simulink model "43_BusNetworkElectricityTransmissionModel"  (R2023b)
settings: Solver=VariableStepAuto  StartTime=0.0  StopTime=0.8  RelTol=1e-3
model workspace (MAT data in the model file):
  BESS_Fp_KDroop = 0.025
  BESS_KSI = 817
  BESS_PWM_fs = 560
  BESS_P_Ki = 0.5
  BESS_P_Kp = 0.0636
  BESS_Pnom = 3000000
  BESS_Q_Ki = 1
  BESS_Q_Kp = 0.0257
  BESS_Vd_Ki = 850
  BESS_Vd_Kp = 0.216
  BESS_Vnom = 1000
  BESS_Vq_KDroop = 0.025
  BESS_Vq_Ki = 850
  BESS_Vq_Kp = 0.216
  Compensation_Ki = 30
  Compensation_Kp = 3
  DC_Ki = 400
  DC_Kp = 8
  F = 0.01
  Flux_min = 0.5
  Grid_Freq_PWM = 2700
  Grid_Ireg_Ki = 5
  Grid_Ireg_Kp = 0.83
  Grid_Ireg_lim = 1.1
  Grid_Modindex_Upper = 1.1
  Grid_conv_Imax = 0.8
  H = 0.685
  Idref_max = 0.9
  Iqref_Tc = 0.3
  Ki_Var = 0.05
  Ki_Vreg = 20
  Ksh = 1.1
  L_pu = 0.3
  Llr = 0.16
  Lls = 0.18
  Lm = 2.9
  LowLoad_P = 130
  Nb_wt = 6
  P_mech = 1080000
  PeakShav_P = 200
  Pitch_Ki = 0
  Pitch_Kp = 150
  Pitch_Max = 27
  Pitch_Tc = 0.01
  Pitch_rate = 10
  Q_Filt = 50
  R_pu = 0.003
  Rotor_Freq_PWM = 1620
  Rotor_Ireg_Ki = 8
  Rotor_Ireg_Kp = 0.6
  Rotor_Ireg_lim = 0.1
  Rotor_Modindex_Upper = 2
  Rr = 0.016
  Rs = 0.023
  SOCBESS : Simulink.Parameter (value not decoded)
  T_set = 0.0001
  Tp = 5e-05
  Ts = 5e-06
  Var_C_Filt = 720000
  Var_reg_max = 1.1
  Var_reg_min = 0.9
  WT_Coeff = [0.645 116 0.4 5 21 0.00912 0.08 0.035]
  WT_H = 4.32
  WT_IGBTRon = 5.931
  WT_Param = [91.204 10143]
  Wind_Freq_Filt = 10000
  Wind_Freq_nom = 60
  Wind_P_nom = 1200000
  Wind_Rotor_V_nom = 1950
  Wind_V_nom = 500
  Zeta_Filt = 0.707106781187
  init = [-0.2 0 0 0 0 0 0 0]
  p = 3
  torque0 = 0.83
  v_Ki = 0.1
  v_Kp = 3.6
  v_Max = 1.2
  v_Min = 0.7
  v_T = 5
  vreg_max = 1
  wind_VDC_nom = 1150
  wt0 = 1.2
undefined symbols (not defined in the file): D1, D11, Delta, DiscIntNeverNeededParam, Iabc, Ion, Lithium, P, Q, Vabc
libraries: powerlib_extras x156, spsSeriesRLCBranchLib x66, spsLoadFlowBusLib x43, spsThreePhaseSeriesRLCLoadLib x33, spsThreePhaseTransformerTwoWindingsLib x32, spsThreePhaseVIMeasurementLib x30, simulink_extras x30, spsDistributedParametersLineLib x22, spsGenericPowerSystemStabilizerLib x20, spsSynchronousMachinepuStandardLib x10, spsExcitationSystemLib x10, spsHydraulicTurbineandGovernorLib x10
(part 5 of 19)

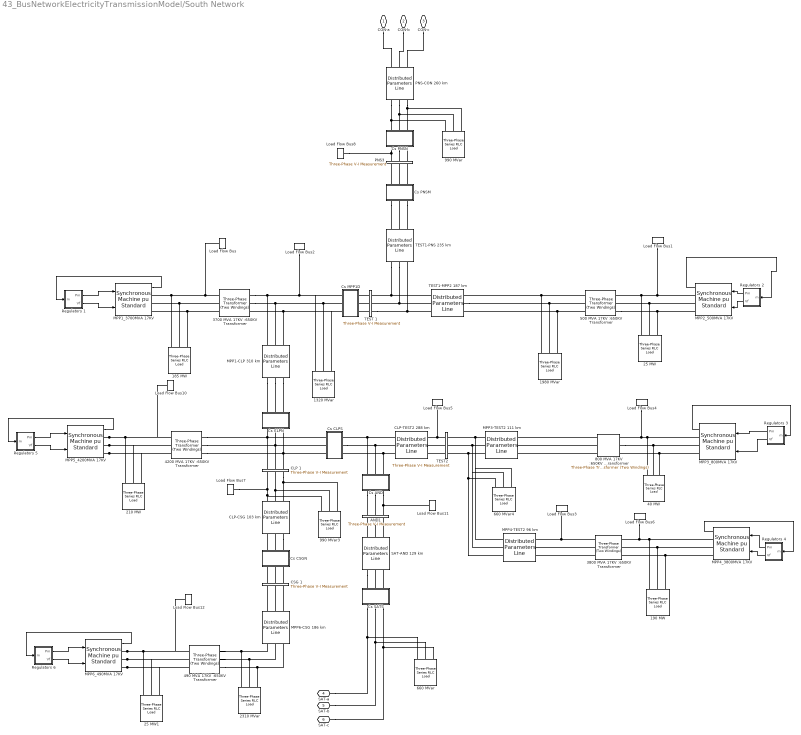
== system 43_BusNetworkElectricityTransmissionModel/South Network ==
  " SAT-AND 129 km" : spsDistributedParametersLineLib/Distributed Parameters Line  Phases=3  Length=129  Frequency=60  Resistance=[0.01273 0.3864]/6  Inductance="[0.9337e-3  4.1264e-3]/6"  Capacitance=[12.74e-9 7.751e-9]*6  x1=[-0.00078 2.60302457371263e-08 -160778.939869371 -239310.302920162;-0.00072 2.65712134423961e-08 -155325.195833165 -242885.5399717;-0.00066 2.70985868238892e-08 -149791.98455669 -246336.512292981;-0.0006 2.76120960676389e-08 -144182.136933079 -249661.454302796;-0.00054 2.81114784528276e-08 -138498.523064033 -252858.664899377;-0.00048 2.85964784861993e-08 -132744.050791429 -255926.508330705;-0.00042 2.90668480327754e-08 -126921.664209612 -258863.415031392;-0.00036 2.95223464428043e-08 -121034.342159143 -261667.882425704;-0.0003 2.99627406748828e-08 -115085.096702768 -264338.4756963;-0.00024 3.03878054151842e-08 -109076.971584392 -266873.828518316;-0.00018 3.07973231927332e-08 -103013.040671842 -269272.643758401;-0.00012 3.11910844906677e-08 -96896.4063842224 -271533.694138353;-6e-05 3.15688878534317e-08 -90730.1981046569 -273655.822863018]  x2=[-0.00078 5.55178195316479e-08 -88962.2973602101 -231944.533349288;-0.00072 5.76982364407432e-08 -83693.5243512018 -233897.335995697;-0.00066 5.98491338659346e-08 -78381.9321886569 -235730.472443085;-0.0006 6.19694113683554e-08 -73030.2383812726 -237443.004824972;-0.00054 6.4057984174857e-08 -67641.1809544889 -239034.056978149;-0.00048 6.61137837329993e-08 -62217.5170496635 -240502.814890934;-0.00042 6.81357582577416e-08 -56762.021513468 -241848.52711964;-0.00036 7.01228732695551e-08 -51277.4854782247 -243070.505173024;-0.0003 7.20741121236823e-08 -45766.7149339116 -244168.123864536;-0.00024 7.39884765302704e-08 -40232.5292925668 -245140.82163217;-0.00018 7.58649870651158e-08 -34677.7599458242 -245988.100825776;-0.00012 7.7702683670755e-08 -29105.2488163219 -246709.527961661;-6e-05 7.95006261476476e-08 -23517.8469037221 -247304.733944374]  x3=[-0.00078 -1.62971978119486e-09 -2676.70735567061 -14439.1653842091;-0.00072 -1.59483091706544e-09 -2349.44448965774 -14496.0134442237;-0.00066 -1.55912610796977e-09 -2020.97960443123 -14545.4450759047;-0.0006 -1.52262362114792e-09 -1691.48074869568 -14587.4349891159;-0.00054 -1.48534213194664e-09 -1361.11650015412 -14621.9617010419;-0.00048 -1.4473007142647e-09 -1030.05587926054 -14649.0075471789;-0.00042 -1.40851883079429e-09 -698.468262745896 -14668.5586903722;-0.00036 -1.36901632306361e-09 -366.523296961816 -14680.6051278957;-0.0003 -1.32881340128554e-09 -34.3908110864396 -14685.1406965693;-0.00024 -1.28793063401772e-09 297.759269763359 -14682.1630759124;-0.00018 -1.24638893763932e-09 629.757011468787 -14671.6737893307;-0.00012 -1.2042095656498e-09 961.432557850576 -14653.678203337;-6e-05 -1.16141409779526e-09 1292.61621757054 -14628.1855248057]  x4=[-0.00078 2.13998612808817e-09 -3708.50494908711 4506.04674626499;-0.00072 2.12843326610419e-09 -3809.4714718435 4421.01671562987;-0.00066 2.11579145833235e-09 -3908.48899860396 4333.72481115204;-0.0006 2.1020671725551e-09 -4005.50687017216 4244.2156929828;-0.00054 2.08726743037064e-09 -4100.47545041233 4152.53515564094;-0.00048 2.07139980360052e-09 -4193.34615164399 4058.73010458342;-0.00042 2.05447241041582e-09 -4284.07145950033 3962.84853220769;-0.00036 2.03649391118366e-09 -4372.60495723746 3864.93949329786;-0.0003 2.01747350403647e-09 -4458.90134948202 3765.05307992739;-0.00024 1.99742092016598e-09 -4542.91648540516 3663.24039583105;-0.00018 1.97634641884464e-09 -4624.60738131092 3559.5535302593;-0.00012 1.95426078217673e-09 -4703.93224262748 3454.04553132848;-6e-05 1.93117530958208e-09 -4780.85048529004 3346.77037888041]  x5=0.000729548621424508  V1=[2.188e-18 3.182e-07 3.182e-07;377 377 377;0.6306 1.295 -0.2758]  V2=[1.209e-19 1.011e-07 1.011e-07;377 377 377;-2.255 -1.798 2.915]  I1=[1.016e-20 9.164e-09 9.164e-09;377 377 377;2.19 2.786 1.215]  I2=[1.089e-20 9.22e-09 9.22e-09;377 377 377;-0.7019 -0.2685 -1.839]  nHarmo=1  Measurements=None  Decoupling=off  VsMag0=0  VrMag0=0  VsAngle0=0  VrAngle0=0  IsMag0=0  IrMag0=0  IsAngle0=0  IrAngle0=0
      settings: LibrarySourceBlock=sps_lib/Power Grid Elements/Distributed Parameters Line
  1320 MVar : spsThreePhaseSeriesRLCLoadLib/Three-Phase Series RLC Load  LConnTagsString=A|B|C  Configuration=Y (grounded)  NominalVoltage=650e3  Vabc=[1e3 1e3 1e3]  Vabcp=[1e3 1e3 1e3]  NominalFrequency=60  UnbalancedPower=off  ActivePower=4400e3  InductivePower=1320e6  CapacitivePower=0  Pabc=[10e3 9e3 11e3]  QLabc=[100 90 110]  QCabc=[100 90 110]  Pabcp=[10e3 9e3 11e3]  QLabcp=[100 90 110]  QCabcp=[100 90 110]  Measurements=None  LoadType=constant Z
  185 MW : spsThreePhaseSeriesRLCLoadLib/Three-Phase Series RLC Load  LConnTagsString=A|B|C  Configuration=Y (grounded)  NominalVoltage=17e3  Vabc=[1e3 1e3 1e3]  Vabcp=[1e3 1e3 1e3]  NominalFrequency=60  UnbalancedPower=off  ActivePower=185e6  InductivePower=0  CapacitivePower=0  Pabc=[10e3 9e3 11e3]  QLabc=[100 90 110]  QCabc=[100 90 110]  Pabcp=[10e3 9e3 11e3]  QLabcp=[100 90 110]  QCabcp=[100 90 110]  Measurements=None  LoadType=constant Z
  190 MW : spsThreePhaseSeriesRLCLoadLib/Three-Phase Series RLC Load  LConnTagsString=A|B|C  Configuration=Y (grounded)  NominalVoltage=17e3  Vabc=[1e3 1e3 1e3]  Vabcp=[1e3 1e3 1e3]  NominalFrequency=60  UnbalancedPower=off  ActivePower=190e6  InductivePower=0  CapacitivePower=0  Pabc=[10e3 9e3 11e3]  QLabc=[100 90 110]  QCabc=[100 90 110]  Pabcp=[10e3 9e3 11e3]  QLabcp=[100 90 110]  QCabcp=[100 90 110]  Measurements=None  LoadType=constant Z
  1980 MVar : spsThreePhaseSeriesRLCLoadLib/Three-Phase Series RLC Load  LConnTagsString=A|B|C  Configuration=Y (grounded)  NominalVoltage=650e3  Vabc=[1e3 1e3 1e3]  Vabcp=[1e3 1e3 1e3]  NominalFrequency=60  UnbalancedPower=off  ActivePower=4400e3  InductivePower=1320e6  CapacitivePower=0  Pabc=[10e3 9e3 11e3]  QLabc=[100 90 110]  QCabc=[100 90 110]  Pabcp=[10e3 9e3 11e3]  QLabcp=[100 90 110]  QCabcp=[100 90 110]  Measurements=None  LoadType=constant Z
  210 MW : spsThreePhaseSeriesRLCLoadLib/Three-Phase Series RLC Load  LConnTagsString=A|B|C  Configuration=Y (grounded)  NominalVoltage=17e3  Vabc=[1e3 1e3 1e3]  Vabcp=[1e3 1e3 1e3]  NominalFrequency=60  UnbalancedPower=off  ActivePower=210e6  InductivePower=0  CapacitivePower=0  Pabc=[10e3 9e3 11e3]  QLabc=[100 90 110]  QCabc=[100 90 110]  Pabcp=[10e3 9e3 11e3]  QLabcp=[100 90 110]  QCabcp=[100 90 110]  Measurements=None  LoadType=constant Z
  2310 MVar : spsThreePhaseSeriesRLCLoadLib/Three-Phase Series RLC Load  LConnTagsString=A|B|C  Configuration=Y (grounded)  NominalVoltage=650e3  Vabc=[1e3 1e3 1e3]  Vabcp=[1e3 1e3 1e3]  NominalFrequency=60  UnbalancedPower=off  ActivePower=7700e3  InductivePower=2310e6  CapacitivePower=0  Pabc=[10e3 9e3 11e3]  QLabc=[100 90 110]  QCabc=[100 90 110]  Pabcp=[10e3 9e3 11e3]  QLabcp=[100 90 110]  QCabcp=[100 90 110]  Measurements=None  LoadType=constant Z
  25 MW : spsThreePhaseSeriesRLCLoadLib/Three-Phase Series RLC Load  LConnTagsString=A|B|C  Configuration=Y (grounded)  NominalVoltage=17e3  Vabc=[1e3 1e3 1e3]  Vabcp=[1e3 1e3 1e3]  NominalFrequency=60  UnbalancedPower=off  ActivePower=25e6  InductivePower=0  CapacitivePower=0  Pabc=[10e3 9e3 11e3]  QLabc=[100 90 110]  QCabc=[100 90 110]  Pabcp=[10e3 9e3 11e3]  QLabcp=[100 90 110]  QCabcp=[100 90 110]  Measurements=None  LoadType=constant Z
  25 MW1 : spsThreePhaseSeriesRLCLoadLib/Three-Phase Series RLC Load  LConnTagsString=A|B|C  Configuration=Y (grounded)  NominalVoltage=17e3  Vabc=[1e3 1e3 1e3]  Vabcp=[1e3 1e3 1e3]  NominalFrequency=60  UnbalancedPower=off  ActivePower=25e6  InductivePower=0  CapacitivePower=0  Pabc=[10e3 9e3 11e3]  QLabc=[100 90 110]  QCabc=[100 90 110]  Pabcp=[10e3 9e3 11e3]  QLabcp=[100 90 110]  QCabcp=[100 90 110]  Measurements=None  LoadType=constant Z
  "3700 MVA 17KV :650KV Transformer " : spsThreePhaseTransformerTwoWindingsLib/Three-Phase Transformer (Two Windings)  Winding1Connection=Delta (D1)  Winding2Connection=Yg  CoreType=Three single-phase transformers  SetSaturation=off  Hysteresis=off  DataFile='hysteresis'  SetInitialFlux=off  Measurements=None  UNITS=pu  NominalPower=[ 3700e6 , 60 ]  Winding1=[ 17e3 , 0.002 , 0.08 ]  Winding2=[ 650e3 , 0.002 , 0.08 ]  Rm=500  Lm=500  L0=0.5  Saturation=[ 0,0 ; 0.0024,1.2 ; 1.0,1.52 ]  InitialFluxes=[ 0.8 , -0.8 , 0.7 ]  BreakLoop=off  DiscreteSolver=Trapezoidal iterative  DataType=off  TransfoNumber=1
  3800 MVA 17KV :650KV Transformer : spsThreePhaseTransformerTwoWindingsLib/Three-Phase Transformer (Two Windings)  Winding1Connection=Yg  Winding2Connection=Delta (D1)  CoreType=Three single-phase transformers  SetSaturation=off  Hysteresis=off  DataFile='hysteresis'  SetInitialFlux=off  Measurements=None  UNITS=pu  NominalPower=[ 3800e6 , 60 ]  Winding1=[ 650e3 , 0.002 , 0.08 ]  Winding2=[ 17e3 , 0.002 , 0.08 ]  Rm=500  Lm=500  L0=0.5  Saturation=[ 0,0 ; 0.0024,1.2 ; 1.0,1.52 ]  InitialFluxes=[ 0.8 , -0.8 , 0.7 ]  BreakLoop=off  DiscreteSolver=Trapezoidal iterative  DataType=off  TransfoNumber=1
  40 MW : spsThreePhaseSeriesRLCLoadLib/Three-Phase Series RLC Load  LConnTagsString=A|B|C  Configuration=Y (grounded)  NominalVoltage=17e3  Vabc=[1e3 1e3 1e3]  Vabcp=[1e3 1e3 1e3]  NominalFrequency=60  UnbalancedPower=off  ActivePower=40e6  InductivePower=0  CapacitivePower=0  Pabc=[10e3 9e3 11e3]  QLabc=[100 90 110]  QCabc=[100 90 110]  Pabcp=[10e3 9e3 11e3]  QLabcp=[100 90 110]  QCabcp=[100 90 110]  Measurements=None  LoadType=constant Z
  4200 MVA 17KV :650KV Transformer : spsThreePhaseTransformerTwoWindingsLib/Three-Phase Transformer (Two Windings)  Winding1Connection=Delta (D1)  Winding2Connection=Yg  CoreType=Three single-phase transformers  SetSaturation=off  Hysteresis=off  DataFile='hysteresis'  SetInitialFlux=off  Measurements=None  UNITS=pu  NominalPower=[ 4200e6 , 60 ]  Winding1=[ 17e3 , 0.002 , 0.08 ]  Winding2=[ 650e3 , 0.002 , 0.08 ]  Rm=500  Lm=500  L0=0.5  Saturation=[ 0,0 ; 0.0024,1.2 ; 1.0,1.52 ]  InitialFluxes=[ 0.8 , -0.8 , 0.7 ]  BreakLoop=off  DiscreteSolver=Trapezoidal iterative  DataType=off  TransfoNumber=1
  490 MVA 17KV :650KV Transformer : spsThreePhaseTransformerTwoWindingsLib/Three-Phase Transformer (Two Windings)  Winding1Connection=Delta (D1)  Winding2Connection=Yg  CoreType=Three single-phase transformers  SetSaturation=off  Hysteresis=off  DataFile='hysteresis'  SetInitialFlux=off  Measurements=None  UNITS=pu  NominalPower=[ 490e6 , 60 ]  Winding1=[ 17e3 , 0.002 , 0.08 ]  Winding2=[ 650e3 , 0.002 , 0.08 ]  Rm=500  Lm=500  L0=0.5  Saturation=[ 0,0 ; 0.0024,1.2 ; 1.0,1.52 ]  InitialFluxes=[ 0.8 , -0.8 , 0.7 ]  BreakLoop=off  DiscreteSolver=Trapezoidal iterative  DataType=off  TransfoNumber=1
  "500 MVA 17KV :650KV Transformer " : spsThreePhaseTransformerTwoWindingsLib/Three-Phase Transformer (Two Windings)  Winding1Connection=Yg  Winding2Connection=Delta (D1)  CoreType=Three single-phase transformers  SetSaturation=off  Hysteresis=off  DataFile='hysteresis'  SetInitialFlux=off  Measurements=None  UNITS=pu  NominalPower=[ 500e6 , 60 ]  Winding1=[650e3 , 0.002 , 0.08 ]  Winding2=[17e3 , 0.002 , 0.08 ]  Rm=500  Lm=500  L0=0.5  Saturation=[ 0,0 ; 0.0024,1.2 ; 1.0,1.52 ]  InitialFluxes=[ 0.8 , -0.8 , 0.7 ]  BreakLoop=off  DiscreteSolver=Trapezoidal iterative  DataType=off  TransfoNumber=1
  660 MVar : spsThreePhaseSeriesRLCLoadLib/Three-Phase Series RLC Load  LConnTagsString=A|B|C  Configuration=Y (grounded)  NominalVoltage=650e3  Vabc=[1e3 1e3 1e3]  Vabcp=[1e3 1e3 1e3]  NominalFrequency=60  UnbalancedPower=off  ActivePower=2200e3  InductivePower=660e6  CapacitivePower=0  Pabc=[10e3 9e3 11e3]  QLabc=[100 90 110]  QCabc=[100 90 110]  Pabcp=[10e3 9e3 11e3]  QLabcp=[100 90 110]  QCabcp=[100 90 110]  Measurements=None  LoadType=constant Z
  660 MVar4 : spsThreePhaseSeriesRLCLoadLib/Three-Phase Series RLC Load  LConnTagsString=A|B|C  Configuration=Y (grounded)  NominalVoltage=650e3  Vabc=[1e3 1e3 1e3]  Vabcp=[1e3 1e3 1e3]  NominalFrequency=60  UnbalancedPower=off  ActivePower=2200e3  InductivePower=660e6  CapacitivePower=0  Pabc=[10e3 9e3 11e3]  QLabc=[100 90 110]  QCabc=[100 90 110]  Pabcp=[10e3 9e3 11e3]  QLabcp=[100 90 110]  QCabcp=[100 90 110]  Measurements=None  LoadType=constant Z
  800 MVA 17KV :650KV Transformer : spsThreePhaseTransformerTwoWindingsLib/Three-Phase Transformer (Two Windings)  Winding1Connection=Yg  Winding2Connection=Delta (D1)  CoreType=Three single-phase transformers  SetSaturation=off  Hysteresis=off  DataFile='hysteresis'  SetInitialFlux=off  Measurements=None  UNITS=pu  NominalPower=[ 800e6 , 60 ]  Winding1=[650e3 , 0.002 , 0.08 ]  Winding2=[ 17e3 , 0.002 , 0.08 ]  Rm=500  Lm=500  L0=0.5  Saturation=[ 0,0 ; 0.0024,1.2 ; 1.0,1.52 ]  InitialFluxes=[ 0.8 , -0.8 , 0.7 ]  BreakLoop=off  DiscreteSolver=Trapezoidal iterative  DataType=off  TransfoNumber=1
  990 MVar : spsThreePhaseSeriesRLCLoadLib/Three-Phase Series RLC Load  LConnTagsString=A|B|C  Configuration=Y (grounded)  NominalVoltage=650e3  Vabc=[1e3 1e3 1e3]  Vabcp=[1e3 1e3 1e3]  NominalFrequency=60  UnbalancedPower=off  ActivePower=2200e3  InductivePower=660e6  CapacitivePower=0  Pabc=[10e3 9e3 11e3]  QLabc=[100 90 110]  QCabc=[100 90 110]  Pabcp=[10e3 9e3 11e3]  QLabcp=[100 90 110]  QCabcp=[100 90 110]  Measurements=None  LoadType=constant Z
  990 MVar3 : spsThreePhaseSeriesRLCLoadLib/Three-Phase Series RLC Load  LConnTagsString=A|B|C  Configuration=Y (grounded)  NominalVoltage=650e3  Vabc=[1e3 1e3 1e3]  Vabcp=[1e3 1e3 1e3]  NominalFrequency=60  UnbalancedPower=off  ActivePower=3300e3  InductivePower=990e6  CapacitivePower=0  Pabc=[10e3 9e3 11e3]  QLabc=[100 90 110]  QCabc=[100 90 110]  Pabcp=[10e3 9e3 11e3]  QLabcp=[100 90 110]  QCabcp=[100 90 110]  Measurements=None  LoadType=constant Z
  AND1 : spsThreePhaseVIMeasurementLib/Three-Phase V-I Measurement  VoltageMeasurement=no  SetLabelV=off  LabelV=Vabc  Vpu=off  VpuLL=off  CurrentMeasurement=no  SetLabelI=off  LabelI=Iabc  Ipu=off  Pbase=100e6  Vbase=500e3  OutputType=Complex  PhasorSimulation=off  PSBequivalent=0
  CLP 1 : spsThreePhaseVIMeasurementLib/Three-Phase V-I Measurement  VoltageMeasurement=no  SetLabelV=off  LabelV=Vabc  Vpu=off  VpuLL=off  CurrentMeasurement=no  SetLabelI=off  LabelI=Iabc  Ipu=off  Pbase=100e6  Vbase=500e3  OutputType=Complex  PhasorSimulation=off  PSBequivalent=0
  CLP-CSG 103 km : spsDistributedParametersLineLib/Distributed Parameters Line  Phases=3  Length=103  Frequency=60  Resistance=[0.01273 0.3864]/6  Inductance="[0.9337e-3  4.1264e-3]/6"  Capacitance=[12.74e-9 7.751e-9]*6  x1=[-0.0006 -1.59527268806973e-09 -150303.114194882 -256726.621745232;-0.00054 -4.5555615464784e-10 -144458.137768001 -260060.467180281;-0.00048 6.84393449720473e-10 -138539.253888559 -263261.260874957;-0.00042 1.82399290575377e-09 -132549.490766916 -266327.36524406;-0.00036 2.96265917331298e-09 -126491.912876563 -269257.21161194;-0.0003 4.09980968969547e-09 -120369.619386282 -272049.301015058;-0.00024 5.23486266768493e-09 -114185.742574547 -274702.204968884;-0.00018 6.36723739320447e-09 -107943.446227001 -277214.566198735;-0.00012 7.49635452242063e-09 -101645.9240178 -279585.099334182;-6e-05 8.62163637814641e-09 -95296.3978756708 -281812.591566671]  x2=[-0.0006 -6.62555188041309e-09 -152758.038264294 -257440.13396002;-0.00054 -5.34862020729046e-09 -146896.295816657 -260829.321358679;-0.00048 -4.06895208123866e-09 -140959.398509749 -264085.06365696;-0.00042 -2.78720220411649e-09 -134950.383769934 -267205.695156943;-0.00036 -1.50402634284513e-09 -128872.325920185 -270189.61928589;-0.0003 -2.20080993905553e-10 -122728.334607209 -273035.30941308;-0.00024 1.06397695253713e-09 -116521.553210489 -275741.309630862;-0.00018 2.34749054871087e-09 -110255.157234075 -278306.235499524;-0.00012 3.62980312534324e-09 -103932.35268194 -280728.774755595;-6e-05 4.91025862762564e-09 -97556.3744177233 -283007.687983231]  x3=[-0.0006 -3.10136755996927e-10 -3832.37611838276 -5044.64343264437;-0.00054 -3.03943415193697e-10 -3717.29819951733 -5130.0325603726;-0.00048 -2.97594571323025e-10 -3600.31844220527 -5212.79706865085;-0.00042 -2.91093472570749e-10 -3481.49669545193 -5292.89461362735;-0.00036 -2.84443445019116e-10 -3360.89375065854 -5370.28421591808;-0.0003 -2.77647890945102e-10 -3238.57131052013 -5444.9262815725;-0.00024 -2.70710287079736e-10 -3114.59195745735 -5516.7826223306;-0.00018 -2.6363418282935e-10 -2989.01912159808 -5585.81647516069;-0.00012 -2.56423198459628e-10 -2861.91704832549 -5651.99252106807;-6e-05 -2.49081023243419e-10 -2733.35076540882 -5715.27690316486]  x4=[-0.0006 1.49194360434117e-10 -3622.40193894112 -5860.20239923923;-0.00054 1.61805038543303e-10 -3488.93184436457 -5940.63384754699;-0.00048 1.74332934204957e-10 -3353.67674778839 -6018.02595780806;-0.00042 1.8677163791617e-10 -3216.70584821922 -6092.33913478878;-0.00036 1.99114785806281e-10 -3078.08922250021 -6163.53535849466;-0.0003 2.11356062892756e-10 -2937.89778945842 -6231.57820362209;-0.00024 2.23489206312044e-10 -2796.20327362144 -6296.43285819422;-0.00018 2.35508008523777e-10 -2653.07816852177 -6358.0661413714;-0.00012 2.47406320486661e-10 -2508.59569960785 -6416.4465204271;-6e-05 2.59178054804441e-10 -2362.82978678048 -6471.54412688065]  x5=0.000582507814005615  V1=[1.056e-22 6.221e-12 6.221e-12;377 377 377;0.3647 1.373 -0.1974]  V2=[1.588e-22 9.824e-12 9.824e-12;377 377 377;0.3755 1.375 -0.1957]  I1=[3.913e-25 1.044e-13 1.044e-13;377 377 377;-0.5956 0.0636 -1.507]  I2=[3.097e-25 1.021e-13 1.021e-13;377 377 377;1.525 2.624 1.053]  nHarmo=1  Measurements=None  Decoupling=off  VsMag0=0  VrMag0=0  VsAngle0=0  VrAngle0=0  IsMag0=0  IrMag0=0  IsAngle0=0  IrAngle0=0
      settings: LibrarySourceBlock=sps_lib/Power Grid Elements/Distributed Parameters Line
  CLP-TEST2 288 km : spsDistributedParametersLineLib/Distributed Parameters Line  Phases=3  Length=288  Frequency=60  Resistance=[0.01273 0.3864]/6  Inductance="[0.9337e-3  4.1264e-3]/6"  Capacitance=[12.74e-9 7.751e-9]*6  x1=[-0.00168 1.73375699558336e-08 0 0;-0.00162 1.73968903310767e-08 0 0;-0.00156 1.74473101357688e-08 0 0;-0.0015 1.74888035742062e-08 0 0;-0.00144 1.75213494175791e-08 0 0;-0.00138 1.75449310148327e-08 0 0;-0.00132 1.7559536301186e-08 0 0;-0.00126 1.75651578043047e-08 0 0;-0.0012 1.7561792648124e-08 0 0;-0.00114 1.75494425543198e-08 0 0;-0.00108 1.75281138414285e-08 0 0;-0.00102 1.74978174216135e-08 -80528.5316001594 -208092.988989509;-0.00096 1.74585687950832e-08 -75801.3786863165 -209861.139027911;-0.0009 1.741038804216e-08 -71035.4443864893 -211521.920229799;-0.00084 1.73532998130075e-08 -66233.1670407299 -213074.482908821;-0.00078 1.72873333150186e-08 -61397.0035828642 -214518.032745223;-0.00072 1.72125222978725e-08 -56529.4282834793 -215851.831192235;-0.00066 1.71289050362679e-08 -51632.9314840408 -217075.195853926;-0.0006 1.70365243103411e-08 -46710.0183227883 -218187.50083433;-0.00054 1.69354273837782e-08 -41763.2074530599 -219188.177057666;-0.00048 1.68256659796352e-08 -36795.0297547032 -220076.712559487;-0.00042 1.67072962538743e-08 -31808.02703923 -220852.652748612;-0.00036 1.65803787666347e-08 -26804.7507493787 -221515.600639704;-0.0003 1.64449784512479e-08 -21787.7606537492 -222065.21705637;-0.00024 1.63011645810171e-08 -16759.6235371778 -222501.220804697;-0.00018 1.61490107337759e-08 -11722.9118875225 -222823.38881711;-0.00012 1.59885947542438e-08 -6680.20257953099 -223031.556266502;-6e-05 1.58199987142001e-08 -1634.07555646387 -223125.616650559]  x2=[-0.00168 6.70084431517853e-08 0 0;-0.00162 6.59395945819886e-08 0 0;-0.00156 6.483701009718e-08 0 0;-0.0015 6.37012537999556e-08 0 0;-0.00144 6.25329067642232e-08 0 0;-0.00138 6.13325667379151e-08 0 0;-0.00132 6.01008478371682e-08 0 0;-0.00126 5.88383802321319e-08 0 0;-0.0012 5.75458098245606e-08 0 0;-0.00114 5.62237979173587e-08 0 0;-0.00108 5.4873020876246e-08 0 0;-0.00102 5.34941697837161e-08 -161669.133849705 -227606.754656263;-0.00096 5.20879500854663e-08 -156479.86606556 -231205.118597313;-0.0009 5.06550812294781e-08 -151210.54029052 -234685.193727509;-0.00084 4.91962962979346e-08 -145863.852409019 -238045.19957611;-0.00078 4.77123416321621e-08 -140442.53788537 -241283.417102038;-0.00072 4.62039764507878e-08 -134949.37036426 -244398.189573373;-0.00066 4.467197246131e-08 -129387.160251693 -247387.923414962;-0.0006 4.31171134652778e-08 -123758.753277142 -250251.089023728;-0.00054 4.15401949572842e-08 -118067.029037616 -252986.221551242;-0.00048 3.99420237179758e-08 -112314.899524406 -255591.921653162;-0.00042 3.83234174012896e-08 -106505.307633259 -258066.856205169;-0.00036 3.66852041161256e-08 -100641.225658735 -260409.758985014;-0.0003 3.50282220026711e-08 -94725.6537735273 -262619.431320343;-0.00024 3.3353318803593e-08 -88761.6184935207 -264694.742701959;-0.00018 3.16613514303164e-08 -82752.1711293665 -266634.631362213;-0.00012 2.99531855246136e-08 -76700.3862253783 -268438.10481822;-6e-05 2.82296950157251e-08 -70609.359986537 -270104.240379637]  x3=[-0.00168 8.78803308459081e-10 0 0;-0.00162 8.90885042172755e-10 0 0;-0.00156 9.0251098263719e-10 0 0;-0.0015 9.13675181806422e-10 0 0;-0.00144 9.24371927869866e-10 0 0;-0.00138 9.34595748174582e-10 0 0;-0.00132 9.44341412025189e-10 0 0;-0.00126 9.5360393335998e-10 0 0;-0.0012 9.62378573301889e-10 0 0;-0.00114 9.70660842582986e-10 0 0;-0.00108 9.78446503841267e-10 0 0;-0.00102 9.8573157378857e-10 -3978.50053051136 606.974855192686;-0.00096 9.92512325248498e-10 -3991.21061365248 516.83544708457;-0.0009 9.9878528906331e-10 -4001.87871969457 426.431616411703;-0.00084 1.00454725586881e-09 -4010.49939063744 335.80961544433;-0.00078 1.0097952777363e-09 -4017.06821598656 245.015808072647;-0.00072 1.01452666968084e-09 -4021.58183500949 154.096646086183;-0.00066 1.01873901103486e-09 -4024.03793845534 63.0986454082026;-0.0006 1.02243014668671e-09 -4024.4352697362 -27.9316377026977;-0.00054 1.02559818818318e-09 -4022.77362557005 -118.947630471632;-0.00048 1.0282415146957e-09 -4019.05385608476 -209.902767434917;-0.00042 1.03035877384958e-09 -4013.27786438311 -300.750514263826;-0.00036 1.03194888241592e-09 -4005.44860556919 -391.444391572407;-0.0003 1.03301102686579e-09 -3995.57008523649 -481.937998697198;-0.00024 1.03354466378647e-09 -3983.64735741853 -572.185037436666;-0.00018 1.03354952015944e-09 -3969.68652200318 -662.139335738217;-0.00012 1.0330255935001e-09 -3953.6947216118 -751.754871320676;-6e-05 1.03197315185901e-09 -3935.68013794496 -840.985795220135]  x4=[-0.00168 -1.56458438388625e-10 0 0;-0.00162 -1.71339675705458e-10 0 0;-0.00156 -1.86133252478206e-10 0 0;-0.0015 -2.0083160003964e-10 0 0;-0.00144 -2.15427198443552e-10 0 0;-0.00138 -2.29912580312103e-10 0 0;-0.00132 -2.44280334656271e-10 0 0;-0.00126 -2.58523110667447e-10 0 0;-0.0012 -2.72633621478248e-10 0 0;-0.00114 -2.8660464789061e-10 0 0;-0.00108 -3.00429042069267e-10 0 0;-0.00102 -3.1409973119871e-10 -3151.6056227922 -9154.67589815408;-0.00096 -3.27609721101776e-10 -2943.74321752368 -9223.61652916484;-0.0009 -3.40952099817995e-10 -2734.37473883095 -9287.83818752643;-0.00084 -3.54120041139877e-10 -2523.60730349639 -9347.30801625177;-0.00078 -3.67106808105326e-10 -2311.54874403447 -9401.99558947761;-0.00072 -3.79905756444394e-10 -2098.30755352259 -9451.87292803096;-0.00066 -3.92510337978614e-10 -1883.99283009406 -9496.9145137438;-0.0006 -4.04914103971167e-10 -1668.71422112147 -9537.09730250861;-0.00054 -4.17110708426175e-10 -1452.58186711906 -9572.40073606815;-0.00048 -4.29093911335434e-10 -1235.70634539281 -9602.8067525335;-0.00042 -4.40857581870909e-10 -1018.19861346703 -9628.29979562478;-0.00036 -4.52395701521387e-10 -800.169952316444 -9648.86682263009;-0.0003 -4.63702367171656e-10 -581.731909432816 -9664.49731107839;-0.00024 -4.74771794122645e-10 -362.996241755153 -9675.18326412296;-0.00018 -4.85598319050987e-10 -144.074858492809 -9680.91921463278;-0.00012 -4.96176402906477e-10 74.9202361293376 -9681.70222798957;-6e-05 -5.06500633745955e-10 293.877000174313 -9677.53190358923]  x5=0.00162875971294774  V1=[1.245e-23 7.93e-13 7.93e-13;377 377 377;-1.837 -1.972 2.74]  V2=[6.065e-20 5.187e-08 5.187e-08;377 377 377;-2.594 -2.004 2.709]  I1=[1.297e-22 5.199e-10 5.199e-10;377 377 377;2.342 2.744 1.173]  I2=[1.117e-22 5.13e-10 5.13e-10;377 377 377;-1.44 -0.7735 -2.344]  nHarmo=1  Measurements=None  Decoupling=off  VsMag0=0  VrMag0=0  VsAngle0=0  VrAngle0=0  IsMag0=0  IrMag0=0  IsAngle0=0  IrAngle0=0
      settings: LibrarySourceBlock=sps_lib/Power Grid Elements/Distributed Parameters Line
  CSG 1 : spsThreePhaseVIMeasurementLib/Three-Phase V-I Measurement  VoltageMeasurement=no  SetLabelV=off  LabelV=Vabc  Vpu=off  VpuLL=off  CurrentMeasurement=no  SetLabelI=off  LabelI=Iabc  Ipu=off  Pbase=100e6  Vbase=500e3  OutputType=Complex  PhasorSimulation=off  PSBequivalent=0
  Cs AND : Subsystem
  Cs CLPN : Subsystem
  Cs CLPS : Subsystem
  Cs CSGN : Subsystem
  Cs MPP1D : Subsystem
  Cs PNSM : Subsystem
  Cs PNSN : Subsystem
  Cs SATS : Subsystem
  Load Flow Bus : spsLoadFlowBusLib/Load Flow Bus  LConnTagsString=a  Phases=single  Connectors=on one side  ID=BUS_1  Vbase=17e3  Vref=1  Vangle=0  VLF=1  VLFb=1  VLFc=1  angleLF=0  angleLFb=0  angleLFc=0
  Load Flow Bus1 : spsLoadFlowBusLib/Load Flow Bus  LConnTagsString=a  Phases=single  Connectors=on one side  ID=BUS_2  Vbase=17e3  Vref=1  Vangle=0  VLF=1  VLFb=1  VLFc=1  angleLF=0  angleLFb=0  angleLFc=0
  Load Flow Bus10 : spsLoadFlowBusLib/Load Flow Bus  LConnTagsString=a  Phases=single  Connectors=on one side  ID=BUS_5  Vbase=17e3  Vref=1  Vangle=0  VLF=1  VLFb=1  VLFc=1  angleLF=0  angleLFb=0  angleLFc=0
  Load Flow Bus11 : spsLoadFlowBusLib/Load Flow Bus  LConnTagsString=a  Phases=single  Connectors=on one side  ID=BUS_11  Vbase=650e3  Vref=1.031  Vangle=17.31  VLF=1  VLFb=1  VLFc=1  angleLF=0  angleLFb=0  angleLFc=0
  Load Flow Bus12 : spsLoadFlowBusLib/Load Flow Bus  LConnTagsString=a  Phases=single  Connectors=on one side  ID=BUS_6  Vbase=17e3  Vref=1  Vangle=0  VLF=1  VLFb=1  VLFc=1  angleLF=0  angleLFb=0  angleLFc=0
  Load Flow Bus2 : spsLoadFlowBusLib/Load Flow Bus  LConnTagsString=a  Phases=single  Connectors=on one side  ID=BUS_7  Vbase=650e3  Vref=1  Vangle=0  VLF=1  VLFb=1  VLFc=1  angleLF=0  angleLFb=0  angleLFc=0
  Load Flow Bus3 : spsLoadFlowBusLib/Load Flow Bus  LConnTagsString=a  Phases=single  Connectors=on one side  ID=BUS_9  Vbase=650e3  Vref=1.031  Vangle=17.31  VLF=1  VLFb=1  VLFc=1  angleLF=0  angleLFb=0  angleLFc=0
  Load Flow Bus4 : spsLoadFlowBusLib/Load Flow Bus  LConnTagsString=a  Phases=single  Connectors=on one side  ID=BUS_3  Vbase=17e3  Vref=1  Vangle=0  VLF=1  VLFb=1  VLFc=1  angleLF=0  angleLFb=0  angleLFc=0
  Load Flow Bus5 : spsLoadFlowBusLib/Load Flow Bus  LConnTagsString=a  Phases=single  Connectors=on one side  ID=BUS_8  Vbase=650e3  Vref=1.031  Vangle=17.31  VLF=1  VLFb=1  VLFc=1  angleLF=0  angleLFb=0  angleLFc=0
  Load Flow Bus6 : spsLoadFlowBusLib/Load Flow Bus  LConnTagsString=a  Phases=single  Connectors=on one side  ID=BUS_4  Vbase=17e3  Vref=1  Vangle=0  VLF=1  VLFb=1  VLFc=1  angleLF=0  angleLFb=0  angleLFc=0
  Load Flow Bus7 : spsLoadFlowBusLib/Load Flow Bus  LConnTagsString=a  Phases=single  Connectors=on one side  ID=BUS_10  Vbase=650e3  Vref=1.031  Vangle=17.31  VLF=1  VLFb=1  VLFc=1  angleLF=0  angleLFb=0  angleLFc=0
  Load Flow Bus8 : spsLoadFlowBusLib/Load Flow Bus  LConnTagsString=a  Phases=single  Connectors=on one side  ID=BUS_12  Vbase=650e3  Vref=1  Vangle=0  VLF=1  VLFb=1  VLFc=1  angleLF=0  angleLFb=0  angleLFc=0
  MPP1-CLP 310 km : spsDistributedParametersLineLib/Distributed Parameters Line  Phases=3  Length=310  Frequency=60  Resistance=[0.01273 0.3864]/6  Inductance="[0.9337e-3  4.1264e-3]/6"  Capacitance=[12.74e-9 7.751e-9]*6  x1=[-0.0018 3.02088878180448e-08 -241444.76658926 -184929.542891138;-0.00174 2.86710925249426e-08 -237200.334725751 -190343.151436196;-0.00168 2.71186285711239e-08 -232834.546788039 -195659.376907842;-0.00162 2.55522902258334e-08 -228349.636393902 -200875.499426893;-0.00156 2.39728788567114e-08 -223747.89810637 -205988.850328684;-0.0015 2.23812025197985e-08 -219031.686259781 -210996.813528411;-0.00144 2.07780755461193e-08 -214203.413755261 -215896.826859564;-0.00138 1.91643181250561e-08 -209265.55082624 -220686.38338478;-0.00132 1.75407558847242e-08 -204220.623774633 -225363.032678442;-0.00126 1.59082194695658e-08 -199071.21367834 -229924.382080355;-0.0012 1.42675441153766e-08 -193819.955070717 -234368.097919882;-0.00114 1.26195692219841e-08 -188469.534592698 -238691.906709888;-0.00108 1.09651379237948e-08 -183022.689618264 -242893.596309903;-0.00102 9.30509665843128e-09 -177482.206853952 -246971.017057887;-0.00096 7.64029473367885e-09 -171850.920913119 -250922.082870045;-0.0009 5.97158389296427e-09 -166131.712865707 -254744.7723081;-0.00084 4.29981787958786e-09 -160327.508764232 -258437.1296135;-0.00078 2.62585199993275e-09 -154441.278146761 -261997.26570802;-0.00072 9.50542685874315e-10 -148476.032517643 -265423.359160252;-0.00066 -7.25252943386227e-10 -142434.823806768 -268713.657117477;-0.0006 -2.4006775198398e-09 -136320.742808141 -271866.476202463;-0.00054 -4.0748738653148e-09 -130136.917598575 -274880.20337471;-0.00048 -5.7469854300253e-09 -123886.511937312 -277753.296755707;-0.00042 -7.41615673079771e-09 -117572.723647382 -280484.286417794;-0.00036 -9.08153378875182e-09 -111198.78297954 -283071.775136195;-0.0003 -1.07422645662122e-08 -104767.950959609 -285514.439103872;-0.00024 -1.23974994026262e-08 -98283.5177200773 -287811.028608803;-0.00018 -1.40463914492664e-08 -91748.8008168095 -289960.368673362;-0.00012 -1.56880971024937e-08 -85167.143531721 -291961.359655455;-6e-05 -1.73217764353606e-08 -78541.9131622937 -293812.977811123]  x2=[-0.0018 1.40172836384768e-07 -245595.185388284 -150943.284096755;-0.00174 1.40794972772388e-07 -242118.377682287 -156459.455808686;-0.00168 1.41345075850346e-07 -238517.697740434 -161895.579971988;-0.00162 1.41822864175742e-07 -234794.987737117 -167248.875365089;-0.00156 1.42228093303241e-07 -230952.152279562 -172516.60314315;-0.0015 1.42560555910133e-07 -226991.157433394 -177696.068239302;-0.00144 1.42820081902405e-07 -222914.02971677 -182784.620743497;-0.00138 1.43006538501763e-07 -218722.855063565 -187779.657258249;-0.00132 1.43119830313568e-07 -214419.777756175 -192678.622230578;-0.00126 1.43159899375634e-07 -210006.999328464 -197479.009259482;-0.0012 1.43126725187888e-07 -205486.777439412 -202178.362378257;-0.00114 1.43020324722858e-07 -200861.424718064 -206774.277311012;-0.00108 1.42840752416988e-07 -196133.307580338 -211264.402702745;-0.00102 1.42588100142789e-07 -191304.845018327 -215646.441322339;-0.00096 1.42262497161831e-07 -186378.507362697 -219918.151237864;-0.0009 1.41864110058616e-07 -181356.815018822 -224077.346963595;-0.00084 1.41393142655348e-07 -176242.337177294 -228121.900578147;-0.00078 1.40849835907652e-07 -171037.690499482 -232049.742813155;-0.00072 1.40234467781301e-07 -165745.537778798 -235858.864111953;-0.00066 1.39547353109997e-07 -160368.586578361 -239547.315657701;-0.0006 1.38788843434304e-07 -154909.58784576 -243113.210370433;-0.00054 1.37959326821787e-07 -149371.334505616 -246554.723872523;-0.00048 1.37059227668473e-07 -143756.660030675 -249870.095422074;-0.00042 1.3608900648172e-07 -138068.436992144 -253057.628813737;-0.00036 1.35049159644615e-07 -132309.575590037 -256115.693246532;-0.0003 1.33940219162015e-07 -126483.022164258 -259042.724158189;-0.00024 1.32762752388361e-07 -120591.757687202 -261837.224025607;-0.00018 1.31517361737411e-07 -114638.796238634 -264497.763131017;-0.00012 1.30204684374035e-07 -108627.183463628 -267022.980293454;-6e-05 1.28825391888227e-07 -102559.995014364 -269411.583565154]  x3=[-0.0018 -4.46641035986106e-10 -4227.66007727613 -2669.0974802106;-0.00174 -4.2101766512237e-10 -4166.20985824951 -2764.03453688525;-0.00168 -3.95178893841645e-10 -4102.62812927671 -2857.55746241734;-0.00162 -3.69137941736765e-10 -4036.94741994511 -2949.61840875007;-0.00156 -3.42908131840007e-10 -3969.20133371926 -3040.1702758022;-0.0015 -3.16502883806786e-10 -3899.42453074867 -3129.16673556535;-0.00144 -2.89935707049908e-10 -3827.65271013506 -3216.56225580623;-0.00138 -2.63220193827908e-10 -3753.92259166807 -3302.31212336179;-0.00132 -2.36370012290995e-10 -3678.27189703866 -3386.37246701534;-0.00126 -2.09398899488179e-10 -3600.73933054007 -3468.70027994179;-0.0012 -1.82320654339138e-10 -3521.36455926597 -3549.25344171081;-0.00114 -1.55149130574438e-10 -3440.18819281601 -3627.99073983639;-0.00108 -1.2789822964771e-10 -3357.25176251924 -3704.87189086191;-0.00102 -1.00581893623408e-10 -3272.59770018588 -3779.8575609699;-0.00096 -7.32140980437871e-11 -3186.26931639846 -3852.90938610596;-0.0009 -4.58088447787665e-11 -3098.31077835328 -3923.98999160651;-0.00084 -1.8380154862307e-11 -3008.76708726369 -3993.06301132035;-0.00078 9.05793868100628e-12 -2917.68405533664 -4060.09310621429;-0.00072 3.64913980155189e-11 -2825.10828233427 -4125.04598245319;-0.00066 6.39061876765233e-11 -2731.08713173266 -4187.88840894537;-0.0006 9.12882817510618e-11 -2635.66870648977 -4248.58823434427;-0.00054 1.18623671053843e-10 -2538.90182443508 -4307.11440349759;-0.00048 1.458983702946e-10 -2440.83599329349 -4363.43697333575;-0.00042 1.73098425233222e-10 -2341.52138535628 -4417.52712819131;-0.00036 2.00209919819003e-10 -2241.00881181198 -4469.35719454158;-0.0003 2.27218983310351e-10 -2139.34969675047 -4518.90065516689;-0.00024 2.54111797371314e-10 -2036.59605085346 -4566.13216271733;-0.00018 2.80874603141295e-10 -1932.80044478487 -4611.0275526809;-0.00012 3.07493708274343e-10 -1828.01598229469 -4653.56385574654;-6e-05 3.33955493944408e-10 -1722.29627305011 -4693.71930955559]  x4=[-0.0018 1.78470729071436e-09 -7957.60929006136 -2503.52124236362;-0.00174 1.76244496843639e-09 -7898.9495168449 -2682.86282961963;-0.00168 1.73928094674634e-09 -7836.24849509981 -2860.83181467839;-0.00162 1.71522707678571e-09 -7769.53830382741 -3037.33714531868;-0.00156 1.69029566495884e-09 -7698.85307319421 -3212.28851815188;-0.0015 1.66449946663671e-09 -7624.22896707031 -3385.59642482292;-0.00144 1.63785167963103e-09 -7545.70416452731 -3557.1721978044;-0.00138 1.61036593744203e-09 -7463.31884030515 -3726.9280557605;-0.00132 1.5820563022833e-09 -7377.11514425802 -3894.77714845756;-0.00126 1.55293725788728e-09 -7287.13717978967 -4060.63360119826;-0.0012 1.52302370209515e-09 -7193.43098128933 -4224.4125587567;-0.00114 1.49233093923478e-09 -7096.04449057963 -4386.03022879192;-0.00108 1.46087467229079e-09 -6995.02753238873 -4545.40392471756;-0.00102 1.4286709948706e-09 -6890.43178885901 -4702.45210800591;-0.00096 1.39573638297062e-09 -6782.31077310558 -4857.09442990449;-0.0009 1.36208768654688e-09 -6670.71980183792 -5009.25177254393;-0.00084 1.32774212089421e-09 -6555.71596705892 -5158.84628941621;-0.00078 1.29271725783864e-09 -6437.35810685546 -5305.80144520231;-0.00072 1.25703101674729e-09 -6315.70677529584 -5450.04205492911;-0.00066 1.22070165536051e-09 -6190.82421144913 -5591.4943224354;-0.0006 1.18374776045088e-09 -6062.77430754257 -5730.0858781274;-0.00054 1.14618823831385e-09 -5931.62257627308 -5865.74581600434;-0.00048 1.10804230509498e-09 -5797.43611728979 -5998.40472993529;-0.00042 1.06932947695856e-09 -5660.28358286458 -6127.99474916862;-0.00036 1.03006956010278e-09 -5520.23514276837 -6254.44957305596;-0.0003 9.90282640626562e-10 -5377.3624483709 -6377.70450497279;-0.00024 9.49989074253079e-10 -5231.73859598261 -6497.69648541844;-0.00018 9.09209475915427e-10 -5083.4380894572 -6614.36412427852;-0.00012 8.67964709209638e-10 -4932.53680207409 -6727.64773223323;-6e-05 8.26275875720474e-10 -4779.11193772024 -6837.48935129549]  x5=0.0017531788576868  V1=[1.492e-21 4.488e-11 4.488e-11;377 377 377;2.889 -1.992 2.721]  V2=[1.003e-22 1.265e-11 1.265e-11;377 377 377;0.8549 1.122 -0.4483]  I1=[2.499e-24 5.251e-13 5.251e-13;377 377 377;-2.215 -0.7076 -2.278]  I2=[3.136e-24 5.274e-13 5.274e-13;377 377 377;1.561 2.663 1.092]  nHarmo=1  Measurements=None  Decoupling=off  VsMag0=0  VrMag0=0  VsAngle0=0  VrAngle0=0  IsMag0=0  IrMag0=0  IsAngle0=0  IrAngle0=0
      settings: LibrarySourceBlock=sps_lib/Power Grid Elements/Distributed Parameters Line
  MPP1_3700MVA 17KV : spsSynchronousMachinepuStandardLib/Synchronous Machine pu Standard  PresetModel=No  MechanicalLoad=Mechanical power Pm  ShowDetailedParameters=on  RotorType=Salient-pole  Units=per unit standard parameters  MeasurementBus=off  NominalParameters=[3700e6 17000 60]  Reactances1=[ 1.81, 0.3, 0.23, 1.76, 0.65, 0.25, 0.15 ]  Reactances2=[ 1.305, 0.296, 0.252, 0.474, 0.243, 0.18 ]  dAxisTimeConstants=Short-circuit  qAxisTimeConstants=Open-circuit  TimeConstants1="[ 4.4849  0.0681  0.1  ]"  TimeConstants2=[ 8.0, 0.03, 1.0, 0.07 ]  TimeConstants3="[  4.49  0.0681  0.0513  ]"  TimeConstants4=[ 8.0, 0.03, 0.3371, 0.0295 ]  TimeConstants5=[ 1.01, 0.053, 0.1 ]  TimeConstants6=[ 1.3201, 0.023, 1.0, 0.07 ]  TimeConstants7=[0.012 0.003 0.003]  TimeConstants8=[ 1.3201, 0.0231, 0.3371, 0.0295 ]  StatorResistance=2.8544e-3  Mechanical=[3.5 0 32]  PolePairs=20  InitialConditions=[0 -81.9543 0.907703 0.907703 0.907703 -8.76021 -128.76 111.24 1.25655]  SetSaturation=off  Saturation=[0.6404,0.7127,0.8441,0.9214,0.9956,1.082,1.19,1.316,1.457;0.7,0.7698,0.8872,0.9466,0.9969,1.046,1.1,1.151,1.201]  LoadFlowParameters=[1,0,0,0,0]  TsPowergui=0  TsBlock=-1  IterativeModel=Trapezoidal non iterative  IterativeDiscreteModel=Trapezoidal non iterative  BusType=PV  Pref=3000e6  Qref=0  Qmin=-inf  Qmax=inf  PLF=0  QLF=0
  MPP2_500MVA 17KV : spsSynchronousMachinepuStandardLib/Synchronous Machine pu Standard  PresetModel=No  MechanicalLoad=Mechanical power Pm  ShowDetailedParameters=on  RotorType=Salient-pole  Units=per unit standard parameters  MeasurementBus=off  NominalParameters=[500e6 17000 60]  Reactances1=[ 1.81, 0.3, 0.23, 1.76, 0.65, 0.25, 0.15 ]  Reactances2=[ 1.305, 0.296, 0.252, 0.474, 0.243, 0.18 ]  dAxisTimeConstants=Short-circuit  qAxisTimeConstants=Open-circuit  TimeConstants1="[ 4.4849  0.0681  0.1  ]"  TimeConstants2=[ 8.0, 0.03, 1.0, 0.07 ]  TimeConstants3="[  4.49  0.0681  0.0513  ]"  TimeConstants4=[ 8.0, 0.03, 0.3371, 0.0295 ]  TimeConstants5=[ 1.01, 0.053, 0.1 ]  TimeConstants6=[ 1.3201, 0.023, 1.0, 0.07 ]  TimeConstants7=[0.012 0.003 0.003]  TimeConstants8=[ 1.3201, 0.0231, 0.3371, 0.0295 ]  StatorResistance=2.8544e-3  Mechanical=[3.5 0 32]  PolePairs=20  InitialConditions=[0 -81.9543 0.907703 0.907703 0.907703 -8.76021 -128.76 111.24 1.25655]  SetSaturation=off  Saturation=[0.6404,0.7127,0.8441,0.9214,0.9956,1.082,1.19,1.316,1.457;0.7,0.7698,0.8872,0.9466,0.9969,1.046,1.1,1.151,1.201]  LoadFlowParameters=[1,0,0,0,0]  TsPowergui=0  TsBlock=-1  IterativeModel=Trapezoidal non iterative  IterativeDiscreteModel=Trapezoidal non iterative  BusType=PV  Pref=400e6  Qref=0  Qmin=-inf  Qmax=inf  PLF=0  QLF=0
  MPP3-TEST2 111 km : spsDistributedParametersLineLib/Distributed Parameters Line  Phases=3  Length=111  Frequency=60  Resistance=[0.01273 0.3864]/6  Inductance="[0.9337e-3  4.1264e-3]/6"  Capacitance=[12.74e-9 7.751e-9]*6  x1=[-0.00066 -1.0892827537438e-08 0 0;-0.0006 -1.09040774577688e-08 0 0;-0.00054 -1.09097486505879e-08 0 0;-0.00048 -1.09098382144084e-08 0 0;-0.00042 -1.09043461034079e-08 -26721.3791585651 -218459.275461859;-0.00036 -1.08932751274516e-08 -21773.5366418889 -219007.787753152;-0.0003 -1.08766309506556e-08 -16814.554381538 -219444.251613431;-0.00024 -1.08544220884882e-08 -11846.9694844683 -219768.443739722;-0.00018 -1.08266599034136e-08 -6873.3234589035 -219980.198269341;-0.00012 -1.07933585990788e-08 -1896.16091405271 -220079.406864759;-6e-05 -1.07545352130464e-08 3081.97174175873 -220066.018769025]  x2=[-0.00066 1.71289050362679e-08 0 0;-0.0006 1.70365243103411e-08 0 0;-0.00054 1.69354273837782e-08 0 0;-0.00048 1.68256659796352e-08 0 0;-0.00042 1.67072962538743e-08 -31808.02703923 -220852.652748612;-0.00036 1.65803787666347e-08 -26804.7507493787 -221515.600639704;-0.0003 1.64449784512479e-08 -21787.7606537492 -222065.21705637;-0.00024 1.63011645810171e-08 -16759.6235371778 -222501.220804697;-0.00018 1.61490107337759e-08 -11722.9118875225 -222823.38881711;-0.00012 1.59885947542438e-08 -6680.20257953099 -223031.556266502;-6e-05 1.58199987142001e-08 -1634.07555646387 -223125.616650559]  x3=[-0.00066 2.36730444113106e-10 0 0;-0.0006 2.56153638236608e-10 0 0;-0.00054 2.75445779425613e-10 0 0;-0.00048 2.94596997464212e-10 0 0;-0.00042 3.13597494235381e-10 -1334.49537059379 -4012.54757408107;-0.00036 3.32437548733884e-10 -1243.40003525562 -4041.7046345773;-0.0003 3.51107522039715e-10 -1151.66855348401 -4068.79388430037;-0.00024 3.69597862249549e-10 -1059.34785680006 -4093.80146388956;-0.00018 3.87899109363673e-10 -966.485178178072 -4116.71457900507;-0.00012 4.06001900125896e-10 -873.128027880335 -4137.52150687383;-6e-05 4.23896972813961e-10 -779.324169149982 -4156.21160228706]  x4=[-0.00066 -1.89863514880659e-10 0 0;-0.0006 -2.09780001559302e-10 0 0;-0.00054 -2.29589160912859e-10 0 0;-0.00048 -2.49280858209372e-10 0 0;-0.00042 -2.68845018812645e-10 -659.629849960837 -5592.37658989697;-0.00036 -2.88271633336608e-10 -532.975425773836 -5605.86580225872;-0.0003 -3.0755076276631e-10 -406.048321510755 -5616.48695009155;-0.00024 -3.26672543542895e-10 -278.913475423479 -5624.23459941996;-0.00018 -3.45627192609989e-10 -151.635932048449 -5629.10478640341;-0.00012 -3.64405012418887e-10 -24.280808928672 -5631.09501936423;-6e-05 -3.82996395890002e-10 103.08673670161 -5630.20428006248]  x5=0.000627751139365274  V1=[1.134e-27 1.175e-15 1.175e-15;377 377 377;0.8883 -1.731 2.981]  V2=[1.245e-23 7.93e-13 7.93e-13;377 377 377;-1.459 -1.742 2.971]  I1=[6.861e-26 2.027e-14 2.027e-14;377 377 377;-2.79 3.007 1.436]  I2=[6.467e-26 2.017e-14 2.017e-14;377 377 377;0.1116 -0.2797 -1.851]  nHarmo=1  Measurements=None  Decoupling=off  VsMag0=0  VrMag0=0  VsAngle0=0  VrAngle0=0  IsMag0=0  IrMag0=0  IsAngle0=0  IrAngle0=0
      settings: LibrarySourceBlock=sps_lib/Power Grid Elements/Distributed Parameters Line
  MPP3_800MVA 17KV : spsSynchronousMachinepuStandardLib/Synchronous Machine pu Standard  PresetModel=No  MechanicalLoad=Mechanical power Pm  ShowDetailedParameters=on  RotorType=Salient-pole  Units=per unit standard parameters  MeasurementBus=off  NominalParameters=[800e6 17000 60]  Reactances1=[ 1.81, 0.3, 0.23, 1.76, 0.65, 0.25, 0.15 ]  Reactances2=[ 1.305, 0.296, 0.252, 0.474, 0.243, 0.18 ]  dAxisTimeConstants=Short-circuit  qAxisTimeConstants=Open-circuit  TimeConstants1="[ 4.4849  0.0681  0.1  ]"  TimeConstants2=[ 8.0, 0.03, 1.0, 0.07 ]  TimeConstants3="[  4.49  0.0681  0.0513  ]"  TimeConstants4=[ 8.0, 0.03, 0.3371, 0.0295 ]  TimeConstants5=[ 1.01, 0.053, 0.1 ]  TimeConstants6=[ 1.3201, 0.023, 1.0, 0.07 ]  TimeConstants7=[0.012 0.003 0.003]  TimeConstants8=[ 1.3201, 0.0231, 0.3371, 0.0295 ]  StatorResistance=2.8544e-3  Mechanical=[3.5 0 32]  PolePairs=20  InitialConditions=[0 -81.9543 0.907703 0.907703 0.907703 -8.76021 -128.76 111.24 1.25655]  SetSaturation=off  Saturation=[0.6404,0.7127,0.8441,0.9214,0.9956,1.082,1.19,1.316,1.457;0.7,0.7698,0.8872,0.9466,0.9969,1.046,1.1,1.151,1.201]  LoadFlowParameters=[1,0,0,0,0]  TsPowergui=0  TsBlock=-1  IterativeModel=Trapezoidal non iterative  IterativeDiscreteModel=Trapezoidal non iterative  BusType=PV  Pref=699.2e6  Qref=0  Qmin=-inf  Qmax=inf  PLF=0  QLF=0
  MPP4-TEST2 96 km : spsDistributedParametersLineLib/Distributed Parameters Line  Phases=3  Length=96  Frequency=60  Resistance=[0.01273 0.3864]/6  Inductance="[0.9337e-3  4.1264e-3]/6"  Capacitance=[12.74e-9 7.751e-9]*6  x1=[-0.0006 2.93984654802104e-08 -23274.2456788866 -202230.020849067;-0.00054 2.97361345742245e-08 -18694.3499429672 -202704.717235316;-0.00048 3.00585901123298e-08 -14104.8898321852 -203075.706142676;-0.00042 3.03656671203148e-08 -9508.21339913661 -203342.797766365;-0.00036 3.0657208491908e-08 -4906.67238842145 -203505.855457374;-0.0003 3.09330650691567e-08 -302.621033447488 -203564.795792375;-0.00024 3.11930957187387e-08 4301.58514803898 -203519.588616404;-0.00018 3.14371674041688e-08 8903.59055907955 -203370.257058287;-0.00012 3.16651552538629e-08 13501.0407286707 -203116.877518809;-6e-05 3.18769426250243e-08 18091.5835163544 -202759.579631623]  x2=[-0.0006 1.70365243103411e-08 -46710.0183227883 -218187.50083433;-0.00054 1.69354273837782e-08 -41763.2074530599 -219188.177057666;-0.00048 1.68256659796352e-08 -36795.0297547032 -220076.712559487;-0.00042 1.67072962538743e-08 -31808.02703923 -220852.652748612;-0.00036 1.65803787666347e-08 -26804.7507493787 -221515.600639704;-0.0003 1.64449784512479e-08 -21787.7606537492 -222065.21705637;-0.00024 1.63011645810171e-08 -16759.6235371778 -222501.220804697;-0.00018 1.61490107337759e-08 -11722.9118875225 -222823.38881711;-0.00012 1.59885947542438e-08 -6680.20257953099 -223031.556266502;-6e-05 1.58199987142001e-08 -1634.07555646387 -223125.616650559]  x3=[-0.0006 8.34800622585055e-10 -3774.07825395545 -379.529207517553;-0.00054 8.23385269572437e-10 -3764.52839779101 -464.792797336403;-0.00048 8.11548657441495e-10 -3753.05253933778 -549.818590571752;-0.00042 7.99296842021711e-10 -3739.65654985698 -634.563086456686;-0.00036 7.86636091568241e-10 -3724.34728298437 -718.98292814121;-0.0003 7.73572883554962e-10 -3707.13257122377 -803.03492487442;-0.00024 7.60113901360472e-10 -3688.02122193978 -886.676074101685;-0.00018 7.46266030848756e-10 -3667.02301285186 -969.86358346555;-0.00012 7.32036356846247e-10 -3644.14868703177 -1052.5548926991;-6e-05 7.17432159517099e-10 -3619.40994740727 -1134.70769540056]  x4=[-0.0006 -4.72976623503226e-10 1647.27662128247 -8810.02174300431;-0.00054 -4.58875359548384e-10 1846.11578728632 -8770.51145576368;-0.00048 -4.44539326480556e-10 2044.01044634108 -8726.51401280186;-0.00042 -4.29975858879158e-10 2240.85935188253 -8678.05192402366;-0.00036 -4.15192407683316e-10 2436.56179237324 -8625.14998352916;-0.0003 -4.00196536379831e-10 2631.01764282848 -8567.83525692864;-0.00024 -3.84995917133551e-10 2824.12741604204 -8506.13706749528;-0.00018 -3.6959832686216e-10 3015.79231348567 -8440.08698116285;-0.00012 -3.54011643257354e-10 3205.9142758563 -8369.71879037598;-6e-05 -3.38243840754474e-10 3394.3960332449 -8295.06849680134]  x5=0.000542919904315913  V1=[8.106e-27 2.861e-16 2.861e-16;377 377 377;-1.836 -1.712 3.001]  V2=[1.245e-23 7.93e-13 7.93e-13;377 377 377;-1.427 -1.722 2.99]  I1=[7.942e-26 2.345e-14 2.345e-14;377 377 377;-2.756 3.026 1.455]  I2=[7.544e-26 2.335e-14 2.335e-14;377 377 377;0.1775 -0.2404 -1.811]  nHarmo=1  Measurements=None  Decoupling=off  VsMag0=0  VrMag0=0  VsAngle0=0  VrAngle0=0  IsMag0=0  IrMag0=0  IsAngle0=0  IrAngle0=0
      settings: LibrarySourceBlock=sps_lib/Power Grid Elements/Distributed Parameters Line
  MPP4_3800MVA 17KV : spsSynchronousMachinepuStandardLib/Synchronous Machine pu Standard  PresetModel=No  MechanicalLoad=Mechanical power Pm  ShowDetailedParameters=on  RotorType=Salient-pole  Units=per unit standard parameters  MeasurementBus=off  NominalParameters=[3800e6 17000 60]  Reactances1=[ 1.81, 0.3, 0.23, 1.76, 0.65, 0.25, 0.15 ]  Reactances2=[ 1.305, 0.296, 0.252, 0.474, 0.243, 0.18 ]  dAxisTimeConstants=Short-circuit  qAxisTimeConstants=Open-circuit  TimeConstants1="[ 4.4849  0.0681  0.1  ]"  TimeConstants2=[ 8.0, 0.03, 1.0, 0.07 ]  TimeConstants3="[  4.49  0.0681  0.0513  ]"  TimeConstants4=[ 8.0, 0.03, 0.3371, 0.0295 ]  TimeConstants5=[ 1.01, 0.053, 0.1 ]  TimeConstants6=[ 1.3201, 0.023, 1.0, 0.07 ]  TimeConstants7=[0.012 0.003 0.003]  TimeConstants8=[ 1.3201, 0.0231, 0.3371, 0.0295 ]  StatorResistance=2.8544e-3  Mechanical=[3.5 0 32]  PolePairs=20  InitialConditions=[0 -81.9543 0.907703 0.907703 0.907703 -8.76021 -128.76 111.24 1.25655]  SetSaturation=off  Saturation=[0.6404,0.7127,0.8441,0.9214,0.9956,1.082,1.19,1.316,1.457;0.7,0.7698,0.8872,0.9466,0.9969,1.046,1.1,1.151,1.201]  LoadFlowParameters=[1,0,0,0,0]  TsPowergui=0  TsBlock=-1  IterativeModel=Trapezoidal non iterative  IterativeDiscreteModel=Trapezoidal non iterative  BusType=PV  Pref=3200e6  Qref=0  Qmin=-inf  Qmax=inf  PLF=0  QLF=0
  MPP5_4200MVA 17KV : spsSynchronousMachinepuStandardLib/Synchronous Machine pu Standard  PresetModel=No  MechanicalLoad=Mechanical power Pm  ShowDetailedParameters=on  RotorType=Salient-pole  Units=per unit standard parameters  MeasurementBus=off  NominalParameters=[4200e6 17000 60]  Reactances1=[ 1.81, 0.3, 0.23, 1.76, 0.65, 0.25, 0.15 ]  Reactances2=[ 1.305, 0.296, 0.252, 0.474, 0.243, 0.18 ]  dAxisTimeConstants=Short-circuit  qAxisTimeConstants=Open-circuit  TimeConstants1="[ 4.4849  0.0681  0.1  ]"  TimeConstants2=[ 8.0, 0.03, 1.0, 0.07 ]  TimeConstants3="[  4.49  0.0681  0.0513  ]"  TimeConstants4=[ 8.0, 0.03, 0.3371, 0.0295 ]  TimeConstants5=[ 1.01, 0.053, 0.1 ]  TimeConstants6=[ 1.3201, 0.023, 1.0, 0.07 ]  TimeConstants7=[0.012 0.003 0.003]  TimeConstants8=[ 1.3201, 0.0231, 0.3371, 0.0295 ]  StatorResistance=2.8544e-3  Mechanical=[3.5 0 32]  PolePairs=20  InitialConditions=[0 -81.9543 0.907703 0.907703 0.907703 -8.76021 -128.76 111.24 1.25655]  SetSaturation=off  Saturation=[0.6404,0.7127,0.8441,0.9214,0.9956,1.082,1.19,1.316,1.457;0.7,0.7698,0.8872,0.9466,0.9969,1.046,1.1,1.151,1.201]  LoadFlowParameters=[1,0,0,0,0]  TsPowergui=0  TsBlock=-1  IterativeModel=Trapezoidal non iterative  IterativeDiscreteModel=Trapezoidal non iterative  BusType=PV  Pref=3700e6  Qref=0  Qmin=-inf  Qmax=inf  PLF=0  QLF=0
  MPP6-CSG 186 km : spsDistributedParametersLineLib/Distributed Parameters Line  Phases=3  Length=186  Frequency=60  Resistance=[0.01273 0.3864]/6  Inductance="[0.9337e-3  4.1264e-3]/6"  Capacitance=[12.74e-9 7.751e-9]*6  x1=[-0.00108 1.3208602511188e-09 0 0;-0.00102 2.15241599202675e-09 0 0;-0.00096 2.9828705171411e-09 0 0;-0.0009 3.81179895058178e-09 0 0;-0.00084 4.63877719724539e-09 0 0;-0.00078 5.46338215978015e-09 0 0;-0.00072 6.28519195505026e-09 0 0;-0.00066 7.10378612997918e-09 -147479.790877794 -243489.125729421;-0.0006 7.91874587666113e-09 -141934.935872809 -246762.499411221;-0.00054 8.72965424663098e-09 -136317.464331976 -249909.624838677;-0.00048 9.53609636418278e-09 -130630.250257533 -252928.891884266;-0.00042 1.03376596386279e-08 -124876.203333289 -255818.755835178;-0.00036 1.11339339753838e-08 -119058.267435972 -258577.738183618;-0.0003 1.19245119857866e-08 -113179.419129092 -261204.427383236;-0.00024 1.27089891955177e-08 -107242.66614007 -263697.479571302;-0.00018 1.34869642515413e-08 -101251.045821434 -266055.61925625;-0.00012 1.42580391274434e-08 -95207.6235968518 -268277.639970244;-6e-05 1.50218193270696e-08 -89115.4913928026 -270362.404886428]  x2=[-0.00108 -1.15706654736948e-08 0 0;-0.00102 -1.0414591796088e-08 0 0;-0.00096 -9.25318982087872e-09 0 0;-0.0009 -8.08705374277784e-09 0 0;-0.00084 -6.91678017855058e-09 0 0;-0.00078 -5.74296786177657e-09 0 0;-0.00072 -4.56621733652663e-09 0 0;-0.00066 -3.38713065011333e-09 -159471.712517598 -255929.191311244;-0.0006 -2.20631104507246e-09 -153642.425715514 -259470.612162782;-0.00054 -1.02436265053298e-09 -147734.532609448 -262879.283054671;-0.00048 1.58109826866557e-10 -141751.055786679 -266153.460047899;-0.00042 1.34050141235713e-09 -135695.056504511 -269291.468013016;-0.00036 2.52220717255553e-09 -129569.633124079 -272291.701487164;-0.0003 3.70262252495942e-09 -123377.91952517 -275152.625495458;-0.00024 4.88114354726294e-09 -117123.083502869 -277872.776336313;-0.00018 6.05716728633451e-09 -110808.325146863 -280450.762330296;-0.00012 7.23009206669882e-09 -104436.875204209 -282885.264532137;-6e-05 8.39931779836506e-09 -98011.9934264286 -285175.037405524]  x3=[-0.00108 -3.75580041647248e-10 0 0;-0.00102 -3.73192268725395e-10 0 0;-0.00096 -3.70613563743063e-10 0 0;-0.0009 -3.67845246013368e-10 0 0;-0.00084 -3.64888731858814e-10 0 0;-0.00078 -3.61745533886673e-10 0 0;-0.00072 -3.58417260215106e-10 0 0;-0.00066 -3.54905613650424e-10 -5084.2000202287 -3902.98674370372;-0.0006 -3.51212390815896e-10 -4994.62316086027 -4016.98103716396;-0.00054 -3.47339481232569e-10 -4902.49095999273 -4128.92016890031;-0.00048 -3.43288866352547e-10 -4807.85055416243 -4238.74686878458;-0.00042 -3.3906261854525e-10 -4710.75036314976 -4346.40494744774;-0.00036 -3.34662900037148e-10 -4611.24006520665 -4451.83932502745;-0.0003 -3.30091961805528e-10 -4509.37057164025 -4554.99605934796;-0.00024 -3.25352142426851e-10 -4405.19400076582 -4655.82237351785;-0.00018 -3.20445866880291e-10 -4298.76365124197 -4754.26668293173;-0.00012 -3.15375645307076e-10 -4190.13397480212 -4850.27862166189;-6e-05 -3.10144071726251e-10 -4079.36054839599 -4943.80906822636]  x4=[-0.00108 1.62959884800164e-10 0 0;-0.00102 1.75338114845862e-10 0 0;-0.00096 1.87626638672129e-10 0 0;-0.0009 1.9981916924311e-10 0 0;-0.00084 2.11909468634872e-10 0 0;-0.00078 2.23891351226843e-10 0 0;-0.00072 2.35758686866491e-10 0 0;-0.00066 2.47505404005618e-10 -3013.27704502799 -6269.95417016849;-0.0006 2.59125492806681e-10 -2870.69527226304 -6336.5039074725;-0.00054 2.70613008217537e-10 -2726.64479875245 -6399.81177229232;-0.00048 2.81962073013034e-10 -2581.19932338021 -6459.84537515451;-0.00042 2.93166880801918e-10 -2434.43325873906 -6516.57400175854;-0.00036 3.04221698997483e-10 -2286.42169305957 -6569.96862869084;-0.0003 3.1512087175047e-10 -2137.24035179371 -6620.00193827364;-0.00024 3.25858822842705e-10 -1986.9655588722 -6666.64833254124;-0.00018 3.36430058539995e-10 -1835.67419765588 -6709.88394633642;-0.00012 3.46829170402824e-10 -1683.44367160067 -6749.68665952025;-6e-05 3.57050838053408e-10 -1530.35186465661 -6786.0361082892]  x5=0.00105190731461208  V1=[8.574e-27 4.511e-17 4.511e-17;377 377 377;-2.265 1.301 -0.2697]  V2=[1.073e-22 6.76e-12 6.76e-12;377 377 377;0.1921 1.269 -0.3021]  I1=[3.519e-25 1.037e-13 1.037e-13;377 377 377;-1.143 -0.2664 -1.837]  I2=[3.187e-25 1.028e-13 1.028e-13;377 377 377;1.591 2.633 1.062]  nHarmo=1  Measurements=None  Decoupling=off  VsMag0=0  VrMag0=0  VsAngle0=0  VrAngle0=0  IsMag0=0  IrMag0=0  IsAngle0=0  IrAngle0=0
      settings: LibrarySourceBlock=sps_lib/Power Grid Elements/Distributed Parameters Line
  MPP6_490MVA 17KV : spsSynchronousMachinepuStandardLib/Synchronous Machine pu Standard  PresetModel=No  MechanicalLoad=Mechanical power Pm  ShowDetailedParameters=on  RotorType=Salient-pole  Units=per unit standard parameters  MeasurementBus=off  NominalParameters=[490e6 13800 60]  Reactances1=[ 1.81, 0.3, 0.23, 1.76, 0.65, 0.25, 0.15 ]  Reactances2=[ 1.305, 0.296, 0.252, 0.474, 0.243, 0.18 ]  dAxisTimeConstants=Short-circuit  qAxisTimeConstants=Open-circuit  TimeConstants1="[ 4.4849  0.0681  0.1  ]"  TimeConstants2=[ 8.0, 0.03, 1.0, 0.07 ]  TimeConstants3="[  4.49  0.0681  0.0513  ]"  TimeConstants4=[ 8.0, 0.03, 0.3371, 0.0295 ]  TimeConstants5=[ 1.01, 0.053, 0.1 ]  TimeConstants6=[ 1.3201, 0.023, 1.0, 0.07 ]  TimeConstants7=[0.012 0.003 0.003]  TimeConstants8=[ 1.3201, 0.0231, 0.3371, 0.0295 ]  StatorResistance=2.8544e-3  Mechanical=[3.5 0 32]  PolePairs=20  InitialConditions=[0 -81.9543 0.907703 0.907703 0.907703 -8.76021 -128.76 111.24 1.25655]  SetSaturation=off  Saturation=[0.6404,0.7127,0.8441,0.9214,0.9956,1.082,1.19,1.316,1.457;0.7,0.7698,0.8872,0.9466,0.9969,1.046,1.1,1.151,1.201]  LoadFlowParameters=[1,0,0,0,0]  TsPowergui=0  TsBlock=-1  IterativeModel=Trapezoidal non iterative  IterativeDiscreteModel=Trapezoidal non iterative  BusType=PV  Pref=415e6  Qref=0  Qmin=-inf  Qmax=inf  PLF=0  QLF=0
  PNS-CON 260 km : spsDistributedParametersLineLib/Distributed Parameters Line  Phases=3  Length=271  Frequency=60  Resistance=[0.01273 0.3864]/6  Inductance="[0.9337e-3  4.1264e-3]/6"  Capacitance=[12.74e-9 7.751e-9]*6  x1=[-0.00156 1.48126219989527e-08 -222729.791092244 -201960.060987846;-0.0015 1.51200540326052e-08 -218104.961005114 -206946.027248242;-0.00144 1.54197503672282e-08 -213368.544389819 -211826.116097176;-0.00138 1.5711557672639e-08 -208522.964484616 -216597.830791018;-0.00132 1.59953266548283e-08 -203570.700377721 -221258.730032359;-0.00126 1.62709121323414e-08 -198514.285738959 -225806.429219024;-0.0012 1.65381731105557e-08 -193356.307523491 -230238.601664078;-0.00114 1.67969728538163e-08 -188099.40464828 -234552.979786201;-0.00108 1.70471789553925e-08 -182746.266641974 -238747.356269824;-0.00102 1.72886634052195e-08 -177299.63226889 -242819.585194435;-0.00096 1.75213026553906e-08 -171762.288127818 -246767.583132471;-0.0009 1.77449776833668e-08 -166137.067226337 -250589.330215236;-0.00084 1.79595740528706e-08 -160426.847531403 -254282.871166304;-0.00078 1.81649819724343e-08 -154634.550496925 -257846.316301876;-0.00072 1.83610963515705e-08 -148763.139569094 -261277.842497576;-0.00066 1.85478168545393e-08 -142815.618670233 -264575.694121195;-0.0006 1.8725047951681e-08 -136795.030661932 -267738.183930905;-0.00054 1.88926989682916e-08 -130704.455788262 -270763.693938483;-0.00048 1.9050684131013e-08 -124547.01009987 -273650.676237104;-0.00042 1.91989226117168e-08 -118325.843859747 -276397.653793279;-0.00036 1.93373385688572e-08 -112044.139931495 -279003.221202532;-0.0003 1.94658611862728e-08 -105705.112150917 -281466.045408431;-0.00024 1.95844247094178e-08 -99312.0036817557 -283784.866384605;-0.00018 1.96929684790028e-08 -92868.0853564364 -285958.497779395;-0.00012 1.97914369620298e-08 -86376.6540026439 -287985.827522815;-6e-05 1.98797797802033e-08 -79841.0307566066 -289865.818395508]  x2=[-0.00156 1.30999794952957e-08 -257066.441384328 -218306.895219534;-0.0015 1.32704634753731e-08 -252063.09958899 -224065.293488377;-0.00144 1.34341580411266e-08 -246930.797654311 -229709.05581282;-0.00138 1.35909794433915e-08 -241672.161360795 -235235.294739774;-0.00132 1.37408474494407e-08 -236289.881123939 -240641.182943291;-0.00126 1.38836853840332e-08 -230786.710617765 -245923.954671076;-0.0012 1.40194201686422e-08 -225165.465365991 -251080.907159499;-0.00114 1.41479823588438e-08 -219429.021301556 -256109.402016378;-0.00108 1.42693061798459e-08 -213580.313295242 -261006.866570827;-0.00102 1.438332956014e-08 -207622.333654135 -265770.795189487;-0.00096 1.44899941632577e-08 -201558.130590711 -270398.750558448;-0.0009 1.45892454176173e-08 -195390.80666331 -274888.364930228;-0.00084 1.46810325444429e-08 -189123.517188814 -279237.341335158;-0.00078 1.47653085837444e-08 -182759.468628323 -283443.454756547;-0.00072 1.4842030418343e-08 -176301.916946676 -287504.553269051;-0.00066 1.49111587959304e-08 -169754.165946633 -291418.559139628;-0.0006 1.49726583491513e-08 -163119.565578596 -295183.469890554;-0.00054 1.50264976136978e-08 -156401.510226705 -298797.35932392;-0.00048 1.50726490444074e-08 -149603.436972216 -302258.378507116;-0.00042 1.51110890293553e-08 -142728.823835017 -305564.756718775;-0.00036 1.5141797901935e-08 -135781.187994219 -308714.802354709;-0.0003 1.51647599509198e-08 -128764.083988696 -311706.903793365;-0.00024 1.51799634285012e-08 -121681.101898517 -314539.530220358;-0.00018 1.51874005562991e-08 -114535.865508198 -317211.232411669;-0.00012 1.51870675293414e-08 -107332.030452706 -319720.643475088;-6e-05 1.51789645180111e-08 -100073.282347167 -322066.479549548]  x3=[-0.00156 1.51654589879552e-10 -6799.66088516677 -1408.22654729267;-0.0015 1.53753434627049e-10 -6766.07021032642 -1561.65832186928;-0.00144 1.55773616276353e-10 -6729.01788894387 -1714.2911231923;-0.00138 1.57714101265206e-10 -6688.52287767137 -1866.04686150023;-0.00132 1.59573896805629e-10 -6644.60589450497 -2016.84789575324;-0.00126 1.6135205139186e-10 -6597.28940818474 -2166.61707335572;-0.0012 1.63047655287156e-10 -6546.59762669939 -2315.27776962899;-0.00114 1.64659840989233e-10 -6492.556484901 -2462.7539270139;-0.00108 1.66187783674095e-10 -6435.19363123629 -2608.97009398329;-0.00102 1.67630701618033e-10 -6374.53841360113 -2753.85146364438;-0.00096 1.68987856597564e-10 -6310.62186432565 -2897.32391201134;-0.0009 1.70258554267123e-10 -6243.47668429749 -3039.31403592852;-0.00084 1.71442144514302e-10 -6173.13722623146 -3179.74919062486;-0.00078 1.72538021792461e-10 -6099.63947709403 -3318.55752688026;-0.00072 1.73545625430536e-10 -6023.02103969174 -3455.66802778502;-0.00066 1.74464439919885e-10 -5943.32111343291 -3591.01054507336;-0.0006 1.7529399517804e-10 -5860.5804742725 -3724.5158350126;-0.00054 1.760338667892e-10 -5774.84145385038 -3856.1155938295;-0.00048 1.76683676221379e-10 -5686.14791783366 -3985.74249265578;-0.00042 1.77243091020065e-10 -5594.54524347425 -4113.33021197476;-0.00036 1.77711824978309e-10 -5500.08029639297 -4238.81347555169;-0.0003 1.78089638283157e-10 -5402.80140660225 -4362.12808383027;-0.00024 1.78376337638341e-10 -5302.75834377963 -4483.21094677829;-0.00018 1.78571776363174e-10 -5200.00229180462 -4602.00011616573;-0.00012 1.78675854467592e-10 -5094.58582257212 -4718.43481725855;-6e-05 1.78688518703315e-10 -4986.56286909568 -4832.45547991222]  x4=[-0.00156 2.51078800504833e-12 -5379.68802534801 -5935.65482814672;-0.0015 5.35831516658982e-12 -5244.06165133974 -6055.81257114093;-0.00144 8.20310091508184e-12 -5105.75231849152 -6172.8720485252;-0.00138 1.10436898055698e-11 -4964.83078841371 -6286.77337050788;-0.00132 1.38786285402893e-11 -4821.36915916502 -6397.45826306799;-0.00126 1.67064667122001e-11 -4675.44082836584 -6504.87009776928;-0.0012 1.95257575470408e-11 -4527.12045564666 -6608.95392073237;-0.00114 2.2335058643526e-11 -4376.4839244508 -6709.65648075019;-0.00108 2.51329327113047e-11 -4223.60830321106 -6806.92625653226;-0.00102 2.79179483063051e-11 -4068.5718059201 -6900.71348306395;-0.00096 3.06886805630877e-11 -3911.45375211466 -6990.97017706718;-0.0009 3.34437119238325e-11 -3752.33452629429 -7077.65016154954;-0.00084 3.61816328635884e-11 -3591.29553679509 -7160.70908942932;-0.00078 3.89010426114115e-11 -3428.41917413976 -7240.10446622426;-0.00072 4.1600549867026e-11 -3263.78876888503 -7315.79567179253;-0.00066 4.42787735126388e-11 -3097.48854898827 -7387.74398111475;-0.0006 4.69343433195449e-11 -2929.60359671483 -7455.91258410641;-0.00054 4.95659006491617e-11 -2760.21980510846 -7520.26660445062;-0.00048 5.21720991481339e-11 -2589.4238340468 -7580.77311744145;-0.00042 5.47516054371523e-11 -2417.30306590459 -7637.40116682881;-0.00036 5.73030997931357e-11 -2243.94556084724 -7690.12178065628;-0.0003 5.98252768244254e-11 -2069.44001177761 -7738.90798608364;-0.00024 6.23168461386478e-11 -1893.8756989591 -7783.73482318675;-0.00018 6.47765330029027e-11 -1717.34244433821 -7824.57935772744;-0.00012 6.72030789959406e-11 -1539.93056558995 -7861.42069288711;-6e-05 6.9595242651994e-11 -1361.73082990969 -7894.23997995794]  x5=0.00153261764655846  V1=[1.516e-17 3.586e-06 3.586e-06;377 377 377;3.054 -1.986 2.727]  V2=[2.167e-13 0.2213 0.2213;377 377 377;-0.8435 -2.017 2.695]  I1=[4.914e-16 0.002352 0.002352;377 377 377;-2.188 2.73 1.159]  I2=[4.262e-16 0.002322 0.002322;377 377 377;0.3532 -0.7649 -2.336]  nHarmo=1  Measurements=None  Decoupling=off  VsMag0=0  VrMag0=0  VsAngle0=0  VrAngle0=0  IsMag0=0  IrMag0=0  IsAngle0=0  IrAngle0=0
      settings: LibrarySourceBlock=sps_lib/Power Grid Elements/Distributed Parameters Line
  PNS3 : spsThreePhaseVIMeasurementLib/Three-Phase V-I Measurement  VoltageMeasurement=no  SetLabelV=off  LabelV=Vabc  Vpu=off  VpuLL=off  CurrentMeasurement=no  SetLabelI=off  LabelI=Iabc  Ipu=off  Pbase=100e6  Vbase=500e3  OutputType=Complex  PhasorSimulation=off  PSBequivalent=0
  Regulators 1 : Subsystem
  Regulators 2 : Subsystem
  Regulators 3 : Subsystem
  Regulators 4 : Subsystem
  Regulators 5 : Subsystem
  Regulators 6 : Subsystem
  TEST 1 : spsThreePhaseVIMeasurementLib/Three-Phase V-I Measurement  VoltageMeasurement=no  SetLabelV=off  LabelV=Vabc  Vpu=off  VpuLL=off  CurrentMeasurement=no  SetLabelI=off  LabelI=Iabc  Ipu=off  Pbase=100e6  Vbase=500e3  OutputType=Complex  PhasorSimulation=off  PSBequivalent=0
  TEST1-MPP2 187 km : spsDistributedParametersLineLib/Distributed Parameters Line  Phases=3  Length=187  Frequency=60  Resistance=[0.01273 0.3864]/6  Inductance="[0.9337e-3  4.1264e-3]/6"  Capacitance=[12.74e-9 7.751e-9]*6  x1=[-0.00108 1.40111637914813e-08 0 0;-0.00102 1.41367140801777e-08 0 0;-0.00096 1.42550317647342e-08 0 0;-0.0009 1.43660563116372e-08 0 0;-0.00084 1.44697309186769e-08 0 0;-0.00078 1.45660025440087e-08 0 0;-0.00072 1.46548219332903e-08 0 0;-0.00066 1.47361436448808e-08 147217.560357682 224788.764073512;-0.0006 1.48099260730899e-08 152264.096094791 221401.574853437;-0.00054 1.48761314694641e-08 157232.73070682 217901.112496637;-0.00048 1.49347259620992e-08 162120.922148493 214289.167904333;-0.00042 1.49856795729701e-08 166926.169530745 210567.589014122;-0.00036 1.5028966233268e-08 171646.014400223 206738.279854529;-0.0003 1.50645637967375e-08 176278.041997081 202803.199570878;-0.00024 1.50924540510075e-08 180819.88249041 198764.361422954;-0.00018 1.51126227269085e-08 185269.212190689 194623.831754984;-0.00012 1.51250595057733e-08 189623.754738629 190383.728938452;-6e-05 1.51297580247159e-08 193881.282269802 186046.222288309]  x2=[-0.00108 1.66722026591201e-08 0 0;-0.00102 1.69567213746101e-08 0 0;-0.00096 1.72325647181207e-08 0 0;-0.0009 1.74995915631003e-08 0 0;-0.00084 1.7757665293681e-08 0 0;-0.00078 1.80066538745734e-08 0 0;-0.00072 1.8246429918619e-08 0 0;-0.00066 1.84768707519629e-08 148624.601148851 233290.494129173;-0.0006 1.86978584768168e-08 153863.065996444 229869.306420351;-0.00054 1.89092800317773e-08 159022.81165641 226330.513326868;-0.00048 1.91110272496701e-08 164101.19830753 222675.92536066;-0.00042 1.93029969128909e-08 169095.627753353 218907.412276459;-0.00036 1.94850908062127e-08 174003.54475149 215026.902115194;-0.0003 1.96572157670349e-08 178822.438320917 211036.380217566;-0.00024 1.98192837330471e-08 183549.84302664 206937.888208315;-0.00018 1.99712117872832e-08 188183.340241059 202733.522951684;-0.00012 2.01129222005434e-08 192720.559381382 198425.435478626;-6e-05 2.02443424711618e-08 197159.17912246 194015.829886297]  x3=[-0.00108 -2.47934700814281e-11 0 0;-0.00102 -2.14846114291868e-11 0 0;-0.00096 -1.81647608527484e-11 0 0;-0.0009 -1.48356168490115e-11 0 0;-0.00084 -1.1498882669564e-11 0 0;-0.00078 -8.15626544926785e-12 0 0;-0.00072 -4.80947533285737e-12 0 0;-0.00066 -1.46022459999772e-12 1861.64467962336 5502.60629643444;-0.0006 1.88977321074914e-12 1985.62450276876 5459.09298839871;-0.00054 5.23880417860239e-12 2108.58844372842 5412.78670751767;-0.00048 8.58515487743589e-12 2230.47359187803 5363.71114494027;-0.00042 1.19271132523987e-11 2351.21758852362 5311.89140863113;-0.00036 1.52629694958338e-11 2470.75865880542 5257.35401052487;-0.0003 1.85910169220476e-11 2589.03564330301 5200.12685296209;-0.00024 2.19095528404817e-11 2705.9880293256 5140.23921441404;-0.00018 2.52168794268405e-11 2821.55598187148 5077.72173450319;-0.00012 2.85113045917302e-11 2935.68037424067 5012.60639832747;-6e-05 3.17911428463624e-11 3048.30281828527 4944.92652009604]  x4=[-0.00108 2.29034243152376e-10 0 0;-0.00102 2.29866477878296e-10 0 0;-0.00096 2.30581108666689e-10 0 0;-0.0009 2.31177769899239e-10 0 0;-0.00084 2.31656156313035e-10 0 0;-0.00078 2.32016023156747e-10 0 0;-0.00072 2.3225718631585e-10 0 0;-0.00066 2.32379522406813e-10 3416.92922158682 5380.40183421673;-0.0006 2.32382968840234e-10 3537.74721376683 5301.74323289869;-0.00054 2.32267523852852e-10 3656.75522910223 5220.37216177775;-0.00048 2.32033246508457e-10 3773.89238089335 5136.33025179746;-0.00042 2.31680256667666e-10 3889.09873960889 5049.66050035188;-0.00036 2.31208734926606e-10 4002.31536354697 4960.40724928732;-0.0003 2.30618922524511e-10 4113.48432899077 4868.61616221624;-0.00024 2.29911121220304e-10 4222.54875984341 4774.33420115489;-0.00018 2.29085693138212e-10 4329.45285672678 4677.60960249667;-0.00012 2.28143060582494e-10 4434.14192552956 4578.49185233353;-6e-05 2.27083705821383e-10 4536.56240538971 4477.03166113793]  x5=0.00105756273028204  V1=[5.148e-22 3.64e-12 3.64e-12;377 377 377;-2.284 2.392 -2.32]  V2=[4.457e-19 3.159e-07 3.159e-07;377 377 377;1.876 2.36 -2.352]  I1=[1.453e-21 4.823e-09 4.823e-09;377 377 377;0.5394 0.8251 2.396]  I2=[1.317e-21 4.781e-09 4.781e-09;377 377 377;-3.011 -2.56 -0.9894]  nHarmo=1  Measurements=None  Decoupling=off  VsMag0=0  VrMag0=0  VsAngle0=0  VrAngle0=0  IsMag0=0  IrMag0=0  IsAngle0=0  IrAngle0=0
      settings: LibrarySourceBlock=sps_lib/Power Grid Elements/Distributed Parameters Line
  TEST1-PNS 235 km : spsDistributedParametersLineLib/Distributed Parameters Line  Phases=3  Length=235  Frequency=60  Resistance=[0.01273 0.3864]/6  Inductance="[0.9337e-3  4.1264e-3]/6"  Capacitance=[12.74e-9 7.751e-9]*6  x1=[-0.00138 1.51247243921935e-08 -188830.571920576 -202130.177804058;-0.00132 1.5450350375679e-08 -184210.569436566 -206349.382246437;-0.00126 1.57680716744226e-08 -179496.321421412 -210463.01453196;-0.0012 1.60777257363371e-08 -174690.239771508 -214468.970050339;-0.00114 1.63791541366827e-08 -169794.783367033 -218365.199280709;-0.00108 1.66722026591201e-08 -164812.456813941 -222149.708840202;-0.00102 1.69567213746101e-08 -159745.809162558 -225820.562503798;-0.00096 1.72325647181207e-08 -154597.432603445 -229375.882194933;-0.0009 1.74995915631003e-08 -149369.961141179 -232813.848946358;-0.00084 1.7757665293681e-08 -144066.069246755 -236132.703830757;-0.00078 1.80066538745734e-08 -138688.470489268 -239330.748860645;-0.00072 1.8246429918619e-08 -133239.916147611 -242406.347857092;-0.00066 1.84768707519629e-08 -127723.193802863 -245357.927286821;-0.0006 1.86978584768168e-08 -122141.125912111 -248183.977067258;-0.00054 1.89092800317773e-08 -116496.568364435 -250883.051339114;-0.00048 1.91110272496701e-08 -110792.409019774 -253453.769206119;-0.00042 1.93029969128909e-08 -105031.56623145 -255894.815441511;-0.00036 1.94850908062127e-08 -99216.9873530823 -258204.94116093;-0.0003 1.96572157670349e-08 -93351.6472306654 -260382.964461373;-0.00024 1.98192837330471e-08 -87438.5466805852 -262427.771025874;-0.00018 1.99712117872832e-08 -81480.7109543446 -264338.31469361;-0.00012 2.01129222005434e-08 -75481.1881907893 -266113.617995138;-6e-05 2.02443424711618e-08 -69443.0478566236 -267752.772652485]  x2=[-0.00138 1.53756279733524e-08 -236071.210620889 -235637.466128158;-0.00132 1.5645267979338e-08 -230681.267653094 -240916.571518974;-0.00126 1.59069035771341e-08 -225173.303886268 -246072.419540173;-0.0012 1.61604009091343e-08 -219550.137296449 -251102.372364641;-0.00114 1.64056302814196e-08 -213814.64479957 -256003.856575568;-0.00108 1.66424662301117e-08 -207969.76077957 -260774.364483064;-0.00102 1.6870787585563e-08 -202018.475587117 -265411.455407135;-0.00096 1.70904775343493e-08 -195963.834009681 -269912.756926379;-0.0009 1.73014236790332e-08 -189808.93371377 -274275.966091765;-0.00084 1.75035180956695e-08 -183556.923660105 -278498.850604862;-0.00078 1.76966573890201e-08 -177211.002492554 -282579.249959922;-0.00072 1.78807427454539e-08 -170774.416901645 -286515.076549238;-0.00066 1.8055679983501e-08 -164250.459963501 -290304.316731202;-0.0006 1.82213796020379e-08 -157642.469455039 -293945.031860519;-0.00054 1.8377756826078e-08 -150953.826146307 -297435.359280057;-0.00048 1.8524731650144e-08 -144187.952070812 -300773.513273813;-0.00042 1.86622288792002e-08 -137348.308774751 -303957.785980523;-0.00036 1.87901781671233e-08 -130438.395546015 -306986.548267432;-0.0003 1.89085140526936e-08 -123461.747623894 -309858.250563787;-0.00024 1.90171759930854e-08 -116421.934390378 -312571.423653632;-0.00018 1.91161083948421e-08 -109322.557543997 -315124.67942748;-0.00012 1.92052606423189e-08 -102167.249257129 -317516.711592498;-6e-05 1.92845871235787e-08 -94959.6703177065 -319746.296340831]  x3=[-0.00138 1.22865260559964e-10 -7410.79448639823 -431.779978545817;-0.00132 1.25896084732231e-10 -7399.1321923904 -599.283800421287;-0.00126 1.28862498141257e-10 -7383.68436563269 -766.481017630971;-0.0012 1.31762983115129e-10 -7364.45890951873 -933.286088989094;-0.00114 1.34596055712139e-10 -7341.4656601471 -1099.61367393894;-0.00108 1.37360266479997e-10 -7314.71638128906 -1265.37867621469;-0.00102 1.40054201197399e-10 -7284.22475836992 -1430.49628737816;-0.00096 1.42676481597564e-10 -7250.00639146741 -1594.88203020849;-0.0009 1.45225766073385e-10 -7212.07878733031 -1758.45180192213;-0.00084 1.47700750363819e-10 -7170.46135042172 -1921.12191720145;-0.00078 1.50100168221172e-10 -7125.17537299136 -2082.80915100968;-0.00072 1.5242279205893e-10 -7076.24402418207 -2243.43078117036;-0.00066 1.54667433579821e-10 -7023.69233817605 -2402.90463068956;-0.0006 1.56832944383767e-10 -6967.54720138691 -2561.14910979913;-0.00054 1.58918216555427e-10 -6907.83733870408 -2718.08325769954;-0.00048 1.60922183231027e-10 -6844.5932987966 -2873.6267839809;-0.00042 1.62843819144185e-10 -6777.84743848392 -3027.70010970105;-0.00036 1.64682141150461e-10 -6707.63390618149 -3180.22440809962;-0.0003 1.66436208730349e-10 -6633.98862442983 -3331.12164492722;-0.00024 1.68105124470462e-10 -6556.9492715159 -3480.31461836921;-0.00018 1.69688034522671e-10 -6476.55526219616 -3627.72699854363;-0.00012 1.71184129040944e-10 -6392.84772753131 -3773.28336655291;-6e-05 1.7259264259568e-10 -6305.86949384281 -3916.9092530696]  x4=[-0.00138 5.19883810717017e-11 -3413.78555010739 -7747.82875443412;-0.00132 5.48025644958662e-11 -3237.6754368664 -7823.05915486255;-0.00126 5.75887099153995e-11 -3059.90886904653 -7894.28713367384;-0.0012 6.03453918868232e-11 -2880.57679530865 -7961.47624931789;-0.00114 6.30712000407029e-11 -2699.77096525535 -8024.59212660162;-0.00108 6.576473980322e-11 -2517.5838824902 -8083.60247427596;-0.00102 6.84246331096611e-11 -2334.10875729116 -8138.47710155667;-0.00096 7.10495191094614e-11 -2149.43945892252 -8189.18793357045;-0.0009 7.36380548624412e-11 -1963.67046760962 -8235.70902571863;-0.00084 7.61889160258786e-11 -1776.89682620103 -8278.01657695084;-0.00078 7.87007975320678e-11 -1589.21409154288 -8316.08894194212;-0.00072 8.1172414256016e-11 -1400.7182855902 -8349.90664216705;-0.00066 8.36025016729372e-11 -1211.50584628031 -8379.45237586532;-0.0006 8.59898165052058e-11 -1021.6735781934 -8404.71102689361;-0.00054 8.83331373584413e-11 -831.318603025543 -8425.66967245934;-0.00048 9.06312653463954e-11 -640.538309899372 -8442.31758973216;-0.00042 9.28830247043251e-11 -449.430305538069 -8454.64626132999;-0.00036 9.50872633905352e-11 -258.092364327936 -8462.64937967662;-0.0003 9.7242853675784e-11 -66.6223782952135 -8466.32285022882;-0.00024 9.93486927202509e-11 124.881692977284 -8465.66479357119;-0.00018 1.01403703137769e-10 316.321872468107 -8460.67554637766;-0.00012 1.03406833547038e-10 507.600215844019 -8451.35766123931;-6e-05 1.05357059109525e-10 698.618861570131 -8437.71590535832]  x5=0.00132902268243999  V1=[4.457e-19 3.159e-07 3.159e-07;377 377 377;1.774 1.251 -0.3202]  V2=[2.934e-17 4.144e-06 4.144e-06;377 377 377;-1.608 -1.933 2.78]  I1=[7.734e-20 5.426e-08 5.426e-08;377 377 377;-2.952 2.797 1.226]  I2=[6.83e-20 5.366e-08 5.366e-08;377 377 377;-0.313 -0.6082 -2.179]  nHarmo=1  Measurements=None  Decoupling=off  VsMag0=0  VrMag0=0  VsAngle0=0  VrAngle0=0  IsMag0=0  IrMag0=0  IsAngle0=0  IrAngle0=0
      settings: LibrarySourceBlock=sps_lib/Power Grid Elements/Distributed Parameters Line
  TEST2 : spsThreePhaseVIMeasurementLib/Three-Phase V-I Measurement  VoltageMeasurement=no  SetLabelV=off  LabelV=Vabc  Vpu=off  VpuLL=off  CurrentMeasurement=no  SetLabelI=off  LabelI=Iabc  Ipu=off  Pbase=100e6  Vbase=500e3  OutputType=Complex  PhasorSimulation=off  PSBequivalent=0
  CON-a : PMIOPort  Side=Left
  CON-b : PMIOPort  Port=2  Side=Left
  CON-c : PMIOPort  Port=3  Side=Left
  SAT-a : PMIOPort  Port=4  Side=Left
  SAT-b : PMIOPort  Port=5  Side=Left
  SAT-c : PMIOPort  Port=6  Side=Left
  wires:
  Regulators 1/2(Vf) -> MPP1_3700MVA 17KV/2
  Regulators 1/1(Pm) -> MPP1_3700MVA 17KV/1
  Regulators 4/1(Pm) -> MPP4_3800MVA 17KV/1
  Regulators 4/2(Vf) -> MPP4_3800MVA 17KV/2
  MPP1_3700MVA 17KV/1 -> Regulators 1/1(m)
  Regulators 3/1(Pm) -> MPP3_800MVA 17KV/1
  Regulators 2/1(Pm) -> MPP2_500MVA 17KV/1
  MPP4_3800MVA 17KV/1 -> Regulators 4/1(m)
  MPP3_800MVA 17KV/1 -> Regulators 3/1(m)
  Regulators 3/2(Vf) -> MPP3_800MVA 17KV/2
  Regulators 2/2(Vf) -> MPP2_500MVA 17KV/2
  MPP2_500MVA 17KV/1 -> Regulators 2/1(m)
  Regulators 5/1(Pm) -> MPP5_4200MVA 17KV/1
  Regulators 5/2(Vf) -> MPP5_4200MVA 17KV/2
  MPP5_4200MVA 17KV/1 -> Regulators 5/1(m)
  Regulators 6/1(Pm) -> MPP6_490MVA 17KV/1
  Regulators 6/2(Vf) -> MPP6_490MVA 17KV/2
  MPP6_490MVA 17KV/1 -> Regulators 6/1(m)
  connections:
  CLP-CSG 103 km/LConn3 -- Cs CSGN/LConn3
  CLP-TEST2 288 km/RConn1 -- Cs CLPS/LConn1 -- Cs AND/RConn1
  CLP 1/LConn3 -- 4200 MVA 17KV :650KV Transformer/RConn3 -- Cs CLPN/RConn3 -- Cs CLPS/RConn3
  "500 MVA 17KV :650KV Transformer "/LConn3 -- 1980 MVar/LConn3 -- TEST1-MPP2 187 km/LConn1
  CLP-CSG 103 km/RConn1 -- 990 MVar3/LConn1 -- CLP 1/RConn1 -- Load Flow Bus7/LConn1
  MPP3-TEST2 111 km/RConn2 -- 660 MVar4/LConn2 -- MPP4-TEST2 96 km/RConn2 -- TEST2/LConn2
  MPP2_500MVA 17KV/RConn2 -- 25 MW/LConn2 -- "500 MVA 17KV :650KV Transformer "/RConn2
  TEST1-PNS 235 km/LConn2 -- TEST 1/LConn2 -- TEST1-MPP2 187 km/RConn2
  "3700 MVA 17KV :650KV Transformer "/LConn3 -- MPP1_3700MVA 17KV/RConn3 -- 185 MW/LConn3
  "500 MVA 17KV :650KV Transformer "/RConn3 -- 25 MW/LConn3 -- MPP2_500MVA 17KV/RConn3
  40 MW/LConn1 -- MPP3_800MVA 17KV/RConn1 -- 800 MVA 17KV :650KV Transformer/RConn1 -- Load Flow Bus4/LConn1
  MPP4_3800MVA 17KV/RConn1 -- 190 MW/LConn1 -- Load Flow Bus6/LConn1 -- 3800 MVA 17KV :650KV Transformer/RConn1
  "500 MVA 17KV :650KV Transformer "/LConn1 -- 1980 MVar/LConn1 -- TEST1-MPP2 187 km/LConn3
  CLP 1/RConn3 -- 990 MVar3/LConn3 -- CLP-CSG 103 km/RConn3
  Cs CSGN/LConn2 -- CLP-CSG 103 km/LConn2
  MPP4_3800MVA 17KV/RConn3 -- 190 MW/LConn3 -- 3800 MVA 17KV :650KV Transformer/RConn3
  "3700 MVA 17KV :650KV Transformer "/LConn1 -- Load Flow Bus/LConn1 -- 185 MW/LConn1 -- MPP1_3700MVA 17KV/RConn1
  CLP 1/LConn1 -- 4200 MVA 17KV :650KV Transformer/RConn1 -- Cs CLPN/RConn1 -- Cs CLPS/RConn1
  CLP 1/LConn2 -- 4200 MVA 17KV :650KV Transformer/RConn2 -- Cs CLPN/RConn2 -- Cs CLPS/RConn2
  3800 MVA 17KV :650KV Transformer/LConn2 -- MPP4-TEST2 96 km/LConn2
  "3700 MVA 17KV :650KV Transformer "/RConn1 -- MPP1-CLP 310 km/LConn1 -- Cs MPP1D/RConn1 -- 1320 MVar/LConn1 -- Load Flow Bus2/LConn1
  3800 MVA 17KV :650KV Transformer/LConn1 -- Load Flow Bus3/LConn1 -- MPP4-TEST2 96 km/LConn1
  "3700 MVA 17KV :650KV Transformer "/LConn2 -- 185 MW/LConn2 -- MPP1_3700MVA 17KV/RConn2
  MPP3-TEST2 111 km/RConn3 -- 660 MVar4/LConn1 -- MPP4-TEST2 96 km/RConn3 -- TEST2/LConn3
  TEST1-MPP2 187 km/RConn1 -- TEST 1/LConn3 -- TEST1-PNS 235 km/LConn3
  TEST2/RConn3 -- CLP-TEST2 288 km/LConn3
  MPP3-TEST2 111 km/RConn1 -- 660 MVar4/LConn3 -- MPP4-TEST2 96 km/RConn1 -- TEST2/LConn1
  Cs CLPS/LConn2 -- Cs AND/RConn2 -- CLP-TEST2 288 km/RConn2
  CLP-TEST2 288 km/RConn3 -- Cs CLPS/LConn3 -- Cs AND/RConn3
  800 MVA 17KV :650KV Transformer/LConn2 -- MPP3-TEST2 111 km/LConn2
  CSG 1/LConn3 -- Cs CSGN/RConn3
  MPP4_3800MVA 17KV/RConn2 -- 190 MW/LConn2 -- 3800 MVA 17KV :650KV Transformer/RConn2
  800 MVA 17KV :650KV Transformer/RConn2 -- 40 MW/LConn2 -- MPP3_800MVA 17KV/RConn2
  800 MVA 17KV :650KV Transformer/LConn1 -- MPP3-TEST2 111 km/LConn1
  MPP1-CLP 310 km/RConn1 -- Cs CLPN/LConn1
  MPP1-CLP 310 km/RConn3 -- Cs CLPN/LConn3
  TEST1-MPP2 187 km/LConn2 -- 1980 MVar/LConn2 -- "500 MVA 17KV :650KV Transformer "/LConn2
  TEST2/RConn1 -- Load Flow Bus5/LConn1 -- CLP-TEST2 288 km/LConn1
  MPP2_500MVA 17KV/RConn1 -- Load Flow Bus1/LConn1 -- 25 MW/LConn1 -- "500 MVA 17KV :650KV Transformer "/RConn1
  800 MVA 17KV :650KV Transformer/LConn3 -- MPP3-TEST2 111 km/LConn3
  MPP1-CLP 310 km/RConn2 -- Cs CLPN/LConn2
  CLP-CSG 103 km/RConn2 -- 990 MVar3/LConn2 -- CLP 1/RConn2
  CSG 1/LConn2 -- Cs CSGN/RConn2
  MPP3_800MVA 17KV/RConn3 -- 40 MW/LConn3 -- 800 MVA 17KV :650KV Transformer/RConn3
  CSG 1/LConn1 -- Cs CSGN/RConn1
  TEST2/RConn2 -- CLP-TEST2 288 km/LConn2
  3800 MVA 17KV :650KV Transformer/LConn3 -- MPP4-TEST2 96 km/LConn3
  Cs CSGN/LConn1 -- CLP-CSG 103 km/LConn1
  MPP5_4200MVA 17KV/RConn1 -- 210 MW/LConn1 -- 4200 MVA 17KV :650KV Transformer/LConn1 -- Load Flow Bus10/LConn1
  MPP5_4200MVA 17KV/RConn2 -- 210 MW/LConn2 -- 4200 MVA 17KV :650KV Transformer/LConn2
  MPP5_4200MVA 17KV/RConn3 -- 210 MW/LConn3 -- 4200 MVA 17KV :650KV Transformer/LConn3
  MPP6_490MVA 17KV/RConn1 -- 25 MW1/LConn1 -- 490 MVA 17KV :650KV Transformer/LConn1 -- Load Flow Bus12/LConn1
  MPP6_490MVA 17KV/RConn2 -- 25 MW1/LConn2 -- 490 MVA 17KV :650KV Transformer/LConn2
  MPP6_490MVA 17KV/RConn3 -- 25 MW1/LConn3 -- 490 MVA 17KV :650KV Transformer/LConn3
  Cs PNSM/LConn3 -- PNS3/RConn3
  Cs PNSM/LConn1 -- PNS3/RConn1
  Cs PNSM/LConn2 -- PNS3/RConn2
  Cs PNSN/RConn2 -- PNS3/LConn2
  PNS3/LConn3 -- Cs PNSN/RConn3
  Cs PNSN/RConn1 -- PNS3/LConn1 -- Load Flow Bus8/LConn1
  490 MVA 17KV :650KV Transformer/RConn1 -- 2310 MVar/LConn1 -- MPP6-CSG 186 km/LConn1
  490 MVA 17KV :650KV Transformer/RConn2 -- 2310 MVar/LConn2 -- MPP6-CSG 186 km/LConn2
  MPP6-CSG 186 km/RConn1 -- CSG 1/RConn1
  MPP6-CSG 186 km/RConn2 -- CSG 1/RConn2
  MPP6-CSG 186 km/RConn3 -- CSG 1/RConn3
  490 MVA 17KV :650KV Transformer/RConn3 -- 2310 MVar/LConn3 -- MPP6-CSG 186 km/LConn3
  SAT-a/RConn1 -- 660 MVar/LConn1 -- Cs SATS/RConn1
  SAT-b/RConn1 -- 660 MVar/LConn2 -- Cs SATS/RConn2
  SAT-c/RConn1 -- 660 MVar/LConn3 -- Cs SATS/RConn3
  Cs SATS/LConn3 -- " SAT-AND 129 km"/LConn3
  " SAT-AND 129 km"/LConn1 -- Cs SATS/LConn1
  Cs SATS/LConn2 -- " SAT-AND 129 km"/LConn2
  Cs PNSM/RConn1 -- TEST1-PNS 235 km/RConn1
  TEST1-PNS 235 km/RConn2 -- Cs PNSM/RConn2
  Cs PNSM/RConn3 -- TEST1-PNS 235 km/RConn3
  PNS-CON 260 km/LConn1 -- 990 MVar/LConn1 -- Cs PNSN/LConn1
  PNS-CON 260 km/LConn2 -- 990 MVar/LConn2 -- Cs PNSN/LConn2
  PNS-CON 260 km/LConn3 -- 990 MVar/LConn3 -- Cs PNSN/LConn3
  CON-a/RConn1 -- PNS-CON 260 km/RConn1
  CON-b/RConn1 -- PNS-CON 260 km/RConn2
  CON-c/RConn1 -- PNS-CON 260 km/RConn3
  AND1/RConn3 -- " SAT-AND 129 km"/RConn3
  AND1/RConn2 -- " SAT-AND 129 km"/RConn2
  AND1/RConn1 -- " SAT-AND 129 km"/RConn1
  Cs AND/LConn1 -- AND1/LConn1
  Cs AND/LConn3 -- Load Flow Bus11/LConn1 -- AND1/LConn3
  Cs AND/LConn2 -- AND1/LConn2
  TEST1-PNS 235 km/LConn1 -- TEST 1/LConn1 -- TEST1-MPP2 187 km/RConn3
  "3700 MVA 17KV :650KV Transformer "/RConn2 -- Cs MPP1D/RConn2 -- 1320 MVar/LConn2 -- MPP1-CLP 310 km/LConn2
  MPP1-CLP 310 km/LConn3 -- Cs MPP1D/RConn3 -- 1320 MVar/LConn3 -- "3700 MVA 17KV :650KV Transformer "/RConn3
  TEST 1/RConn1 -- Cs MPP1D/LConn1
  TEST 1/RConn2 -- Cs MPP1D/LConn2
  TEST 1/RConn3 -- Cs MPP1D/LConn3
